simulink model "OMAP"  (R2018b)
settings: Solver=FixedStepDiscrete  StartTime=0.0  StopTime=10.0  FixedStep=0.01  RelTol=1e-3
values from neighbouring files (symbols this model uses):
  Clb_ICADirect_LaneDisp_StateFive = Simulink.Parameter    [omap_ver_442.m]
  Clb_ICADirect_LaneDisp_StateFour = Simulink.Parameter    [omap_ver_442.m]
  Clb_ICADirect_LaneDisp_StateOne = Simulink.Parameter    [omap_ver_442.m]
  Clb_ICADirect_LaneDisp_StateThree = Simulink.Parameter    [omap_ver_442.m]
  Clb_ICADirect_LaneDisp_StateTwo = Simulink.Parameter    [omap_ver_442.m]
  Clb_ICADirect_LaneDisp_StateZero = Simulink.Parameter    [omap_ver_442.m]
  Clb_ICADirect_LaneDispSW = Simulink.Parameter    [omap_ver_442.m]
  Clb_ICADirect_TrnLghtsCom_Switch = Simulink.Parameter    [omap_ver_442.m]
  Clb_ICADirect_TrnLghtsCom_Value = Simulink.Parameter    [omap_ver_442.m]
  Clb_ICADirect_TrnLghtsCrtl_Inhb = Simulink.Parameter    [omap_ver_442.m]
  OMAP_ACCAEB_EMSESC_Decel = Simulink.Parameter    [omap_ver_442.m]
  OMAP_ACCFCW_IC_Decel = Simulink.Parameter    [omap_ver_442.m]
  OMAP_clb_ACC_RVVReqType = Simulink.Parameter    [omap_ver_442.m]
  OMAP_clb_ACC_RVVReqType_Switch = Simulink.Parameter    [omap_ver_442.m]
  OMAP_clb_ACCHeadwayDisplay = Simulink.Parameter    [omap_ver_442.m]
  OMAP_clb_ACCHeadwayDisplay_Switch = Simulink.Parameter    [omap_ver_442.m]
  OMAP_clb_ACCHeadwayIcon = Simulink.Parameter    [omap_ver_442.m]
  OMAP_clb_ACCHeadwayIcon_Switch = Simulink.Parameter    [omap_ver_442.m]
  OMAP_clb_ACCMessagePrompt = Simulink.Parameter    [omap_ver_442.m]
  OMAP_clb_ACCMessagePrompt_Switch = Simulink.Parameter    [omap_ver_442.m]
  OMAP_clb_ACCRequestEPB = Simulink.Parameter    [omap_ver_442.m]
  OMAP_clb_ACCRequestEPB_Switch = Simulink.Parameter    [omap_ver_442.m]
  OMAP_clb_ACCSetSpeed = Simulink.Parameter    [omap_ver_442.m]
  OMAP_clb_ACCSetSpeed_Switch = Simulink.Parameter    [omap_ver_442.m]
  OMAP_clb_ACCSetSpeedDis = Simulink.Parameter    [omap_ver_442.m]
  OMAP_clb_ACCSetSpeedDis_Switch = Simulink.Parameter    [omap_ver_442.m]
  OMAP_clb_ACCState = Simulink.Parameter    [omap_ver_442.m]
  OMAP_clb_ACCState_Switch = Simulink.Parameter    [omap_ver_442.m]
  OMAP_clb_ACCStatusIconDis = Simulink.Parameter    [omap_ver_442.m]
  OMAP_clb_ACCStatusIconDis_Switch = Simulink.Parameter    [omap_ver_442.m]
  OMAP_clb_ACCTorqueReq = Simulink.Parameter    [omap_ver_442.m]
  OMAP_clb_ACCTorqueReq_Switch = Simulink.Parameter    [omap_ver_442.m]
  OMAP_clb_ADAS_State = Simulink.Parameter    [omap_ver_442.m]
  OMAP_clb_ADAS_State_Switch = Simulink.Parameter    [omap_ver_442.m]
  OMAP_clb_AEBAlertReq = Simulink.Parameter    [omap_ver_442.m]
  OMAP_clb_AEBAlertReq_Switch = Simulink.Parameter    [omap_ver_442.m]
  OMAP_clb_AEBBrakingProg = Simulink.Parameter    [omap_ver_442.m]
  OMAP_clb_AEBBrakingProg_Switch = Simulink.Parameter    [omap_ver_442.m]
  OMAP_clb_AEBFaultStatus = Simulink.Parameter    [omap_ver_442.m]
  OMAP_clb_AEBFaultStatus_Switch = Simulink.Parameter    [omap_ver_442.m]
  OMAP_clb_AEBMassageDisp = Simulink.Parameter    [omap_ver_442.m]
  OMAP_clb_AEBMassageDisp_Switch = Simulink.Parameter    [omap_ver_442.m]
  OMAP_clb_AEBState = Simulink.Parameter    [omap_ver_442.m]
  OMAP_clb_AEBState_Switch = Simulink.Parameter    [omap_ver_442.m]
  OMAP_clb_AEBSwitchStatus = Simulink.Parameter    [omap_ver_442.m]
  OMAP_clb_AEBSwitchStatus_Switch = Simulink.Parameter    [omap_ver_442.m]
  OMAP_clb_BrakeRequest = Simulink.Parameter    [omap_ver_442.m]
  OMAP_clb_BrakeRequest_Switch = Simulink.Parameter    [omap_ver_442.m]
  OMAP_clb_DecelerationSet = Simulink.Parameter    [omap_ver_442.m]
  OMAP_clb_DecelerationSet_Switch = Simulink.Parameter    [omap_ver_442.m]
  OMAP_clb_DecelerationType = Simulink.Parameter    [omap_ver_442.m]
  OMAP_clb_DecelerationType_Switch = Simulink.Parameter    [omap_ver_442.m]
  OMAP_clb_DeclControlReq = Simulink.Parameter    [omap_ver_442.m]
  OMAP_clb_DeclControlReq_Switch = Simulink.Parameter    [omap_ver_442.m]
  OMAP_clb_DownorUpGearMinTime = Simulink.Parameter    [omap_ver_442.m]
  OMAP_clb_DownorUpGearMinTime_Switch = Simulink.Parameter    [omap_ver_442.m]
  OMAP_clb_ELKPopupMessage = Simulink.Parameter    [omap_ver_442.m]
  OMAP_clb_ELKPopupMessage_Switch = Simulink.Parameter    [omap_ver_442.m]
  OMAP_clb_ELKSts = Simulink.Parameter    [omap_ver_442.m]
  OMAP_clb_ELKSts_Switch = Simulink.Parameter    [omap_ver_442.m]
  OMAP_clb_ESAFaultSt = Simulink.Parameter    [omap_ver_442.m]
  OMAP_clb_ESAFaultSt_Switch = Simulink.Parameter    [omap_ver_442.m]
  OMAP_clb_ESARequest = Simulink.Parameter    [omap_ver_442.m]
  OMAP_clb_ESARequest_Switch = Simulink.Parameter    [omap_ver_442.m]
  OMAP_clb_ESAState = Simulink.Parameter    [omap_ver_442.m]
  OMAP_clb_ESAState_Switch = Simulink.Parameter    [omap_ver_442.m]
  OMAP_clb_ESATorqueReq = Simulink.Parameter    [omap_ver_442.m]
  OMAP_clb_ESATorqueReq_Switch = Simulink.Parameter    [omap_ver_442.m]
  OMAP_clb_ESCDriveOff = Simulink.Parameter    [omap_ver_442.m]
  OMAP_clb_ESCDriveOff_Switch = Simulink.Parameter    [omap_ver_442.m]
  OMAP_clb_ESCHoldReq = Simulink.Parameter    [omap_ver_442.m]
  OMAP_clb_ESCHoldReq_Switch = Simulink.Parameter    [omap_ver_442.m]
  OMAP_clb_Handsoffwarning = Simulink.Parameter    [omap_ver_442.m]
  OMAP_clb_Handsoffwarning_Switch = Simulink.Parameter    [omap_ver_442.m]
  OMAP_clb_HapticAlarmReq = Simulink.Parameter    [omap_ver_442.m]
  OMAP_clb_HapticAlarmReq_Switch = Simulink.Parameter    [omap_ver_442.m]
  OMAP_clb_HMIPopupMassage = Simulink.Parameter    [omap_ver_442.m]
  OMAP_clb_HMIPopupMassage_Switch = Simulink.Parameter    [omap_ver_442.m]
  OMAP_clb_HWAActionSts = Simulink.Parameter    [omap_ver_442.m]
  OMAP_clb_HWAActionSts_Switch = Simulink.Parameter    [omap_ver_442.m]
  OMAP_clb_HWAMode = Simulink.Parameter    [omap_ver_442.m]
  OMAP_clb_HWAMode_Switch = Simulink.Parameter    [omap_ver_442.m]
  OMAP_clb_HWATurnOnIdctr = Simulink.Parameter    [omap_ver_442.m]
  OMAP_clb_HWATurnOnIdctr_Switch = Simulink.Parameter    [omap_ver_442.m]
  OMAP_clb_ICAMassageDisp = Simulink.Parameter    [omap_ver_442.m]
  OMAP_clb_ICAMassageDisp_Switch = Simulink.Parameter    [omap_ver_442.m]
  OMAP_clb_ICAStatusIcon = Simulink.Parameter    [omap_ver_442.m]
  OMAP_clb_ICAStatusIcon_Switch = Simulink.Parameter    [omap_ver_442.m]
  OMAP_clb_ISLCDriverRemind = Simulink.Parameter    [omap_ver_442.m]
  OMAP_clb_ISLCDriverRemind_Switch = Simulink.Parameter    [omap_ver_442.m]
  OMAP_clb_ISLCState = Simulink.Parameter    [omap_ver_442.m]
  OMAP_clb_ISLCState_Switch = Simulink.Parameter    [omap_ver_442.m]
  OMAP_clb_JAFaultSt = Simulink.Parameter    [omap_ver_442.m]
  OMAP_clb_JAFaultSt_Switch = Simulink.Parameter    [omap_ver_442.m]
  OMAP_clb_LCAPopupMessage = Simulink.Parameter    [omap_ver_442.m]
  OMAP_clb_LCAPopupMessage_Switch = Simulink.Parameter    [omap_ver_442.m]
  OMAP_clb_LCAStatusDisplay = Simulink.Parameter    [omap_ver_442.m]
  OMAP_clb_LCAStatusDisplay_Switch = Simulink.Parameter    [omap_ver_442.m]
  OMAP_clb_LDWStatusDisplay = Simulink.Parameter    [omap_ver_442.m]
  OMAP_clb_LDWStatusDisplay_Switch = Simulink.Parameter    [omap_ver_442.m]
  OMAP_clb_LDWWarningSt = Simulink.Parameter    [omap_ver_442.m]
  OMAP_clb_LDWWarningSt_Switch = Simulink.Parameter    [omap_ver_442.m]
  OMAP_clb_LightControlValid = Simulink.Parameter    [omap_ver_442.m]
  OMAP_clb_LightControlValid_Switch = Simulink.Parameter    [omap_ver_442.m]
  OMAP_clb_LKAActivation = Simulink.Parameter    [omap_ver_442.m]
  OMAP_clb_LKAActivation_Switch = Simulink.Parameter    [omap_ver_442.m]
  OMAP_clb_LKAAngleReq = Simulink.Parameter    [omap_ver_442.m]
  OMAP_clb_LKAAngleReq_Switch = Simulink.Parameter    [omap_ver_442.m]
  OMAP_clb_LKAMode = Simulink.Parameter    [omap_ver_442.m]
  OMAP_clb_LKAMode_Switch = Simulink.Parameter    [omap_ver_442.m]
  OMAP_clb_LKAorELK_CoolTime = Simulink.Parameter    [omap_ver_442.m]
  OMAP_clb_LKAState = Simulink.Parameter    [omap_ver_442.m]
  OMAP_clb_LKAState_Switch = Simulink.Parameter    [omap_ver_442.m]
  OMAP_clb_LKAStatusDisplay = Simulink.Parameter    [omap_ver_442.m]
  OMAP_clb_LKAStatusDisplay_Switch = Simulink.Parameter    [omap_ver_442.m]
  OMAP_clb_LKASwitchState = Simulink.Parameter    [omap_ver_442.m]
  OMAP_clb_LKASwitchState_Switch = Simulink.Parameter    [omap_ver_442.m]
  OMAP_clb_LKATorqFactReq = Simulink.Parameter    [omap_ver_442.m]
  OMAP_clb_LKATorqFactReq_Switch = Simulink.Parameter    [omap_ver_442.m]
  OMAP_clb_PrefillRequest = Simulink.Parameter    [omap_ver_442.m]
  ... (+36 more)
libraries: simulink x184, canmsglib x2
(part 3 of 14)

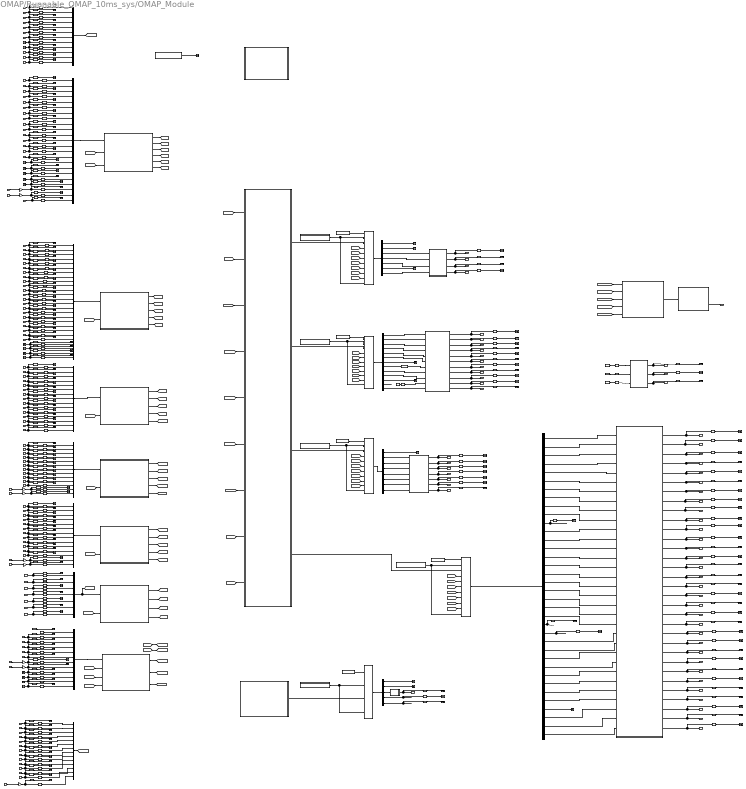
== system OMAP/Runnable_OMAP_10ms_sys/OMAP_Module ==
  note: 暂未参与运算的输出接口
  note: 仲裁#12——ACC单功能调试模式
      | EMS、ESC、EPS、IC：只体现本功能的信号、且其他信号内容强制为“不动作”
  note: 仲裁#17——ESA单功能调试模式
      | EMS、ESC、EPS、IC：只体现本功能的信号、且其他信号内容强制为“不动作”
  note: 仲裁#13——AEB单功能调试模式
      | EMS、ESC、EPS、IC：只体现本功能的信号、且其他信号内容强制为“不动作”
  note: 上面这是版本号
      | 蓝色的子系统是输入，橙色是仲裁输出，
      | 翠绿色的模块是标定量
  note: 仲裁#18——ICA单功能调试模式
      | EMS、ESC：只体现ACC的信号、且其他信号内容强制为“不动作”
      | EPS：只体现本功能的信号、且其他信号内容强制为“不动作”
      | IC：只体现本功能及ACC综合后的的信号、且其他信号内容强制为“不动作”
  note: 仲裁#16——ELK单功能调试模式
      | EMS、ESC、EPS、IC：只体现本功能的信号、且其他信号内容强制为“不动作”
  note: 仲裁#15——LKA单功能调试模式
      | EMS、ESC、EPS、IC：只体现本功能的信号、且其他信号内容强制为“不动作”
  note: 仲裁#14——JA单功能调试模式——
      | EMS、ESC、EPS、IC：只体现本功能的信号、且其他信号内容强制为“不动作”
  FDMMve_d_JaFcnConf : Inport  OutDataTypeStr=uint16
  FDMMve_d_AebFcnConf : Inport  Port=2  OutDataTypeStr=uint16
  FDMMve_d_EsaFcnConf : Inport  Port=3  OutDataTypeStr=uint16
  FDMMve_d_ElkFcnConf : Inport  Port=4  OutDataTypeStr=uint16
  FDMMve_d_LkaFcnConf : Inport  Port=5  OutDataTypeStr=uint16
  FDMMve_d_IcaFcnConf : Inport  Port=6  OutDataTypeStr=uint16
  FDMMve_d_AccFcnConf : Inport  Port=7  OutDataTypeStr=uint16
  FDMMve_d_EwFcnConf : Inport  Port=8  OutDataTypeStr=uint16
  FDMMve_g_Adas2Fapa : Inport  Port=9  OutDataTypeStr=uint32
  FDMMve_d_SignalTStamp : Inport  Port=10  OutDataTypeStr=uint16
  ACCSve_d_ACC_State : Inport  Port=11  OutDataTypeStr=uint16
  ACCSve_g_ACC_TqReq : Inport  Port=12  OutDataTypeStr=single
  ACCSve_d_ACC_TqFlag : Inport  Port=13  OutDataTypeStr=uint16
  ACCSve_g_ACC_DecReq : Inport  Port=14  OutDataTypeStr=single
  ACCSve_d_ACC_DecFlag : Inport  Port=15  OutDataTypeStr=uint16
  ACCSve_d_CIPV_ID : Inport  Port=16  OutDataTypeStr=uint16
  ACCSve_d_ACCActive_Signal : Inport  Port=17  OutDataTypeStr=uint16
  ACCSve_d_ACC_go_request : Inport  Port=18  OutDataTypeStr=uint16
  ACCSve_d_VelocitySet : Inport  Port=19  OutDataTypeStr=uint16
  ACCSve_d_HeadWaySet : Inport  Port=20  OutDataTypeStr=uint16
  ACCSve_d_SignalTStamp : Inport  Port=21  OutDataTypeStr=uint16
  ACCSve_d_ACC_ICA_Flag : Inport  Port=22  OutDataTypeStr=uint16
  ACCSve_d_ACC_ESCDriveOff : Inport  Port=23  OutDataTypeStr=uint16
  ACCSve_d_ACC_ESCHoldReq : Inport  Port=24  OutDataTypeStr=uint16
  ACCSve_d_ACC_EPBReq : Inport  Port=25  OutDataTypeStr=uint16
  ACCSve_d_ACCMessagePrompt : Inport  Port=26  OutDataTypeStr=uint16
  ACCSve_d_ACC_ISLCState : Inport  Port=27  OutDataTypeStr=uint16
  ACCSve_d_ACC_ISLCDriverRemind : Inport  Port=28  OutDataTypeStr=uint16
  AEBSve_d_Prefill_request : Inport  Port=29  OutDataTypeStr=uint16
  AEBSve_d_functionFARCState : Inport  Port=30  OutDataTypeStr=uint16
  AEBSve_g_DecSetpoint : Inport  Port=31  OutDataTypeStr=single
  AEBSve_d_MDDdecRequest : Inport  Port=32  OutDataTypeStr=uint16
  AEBSve_d_MDDdecType : Inport  Port=33  OutDataTypeStr=uint16
  AEBSve_d_ESCDriveOff : Inport  Port=34  OutDataTypeStr=uint16
  AEBSve_d_ESCHoldReq : Inport  Port=35  OutDataTypeStr=uint16
  AEBSve_d_HapticAlarm : Inport  Port=36  OutDataTypeStr=uint16
  AEBSve_d_Braking_progress : Inport  Port=37  OutDataTypeStr=uint16
  AEBSve_d_AEBStatus : Inport  Port=38  OutDataTypeStr=uint16
  AEBSve_d_FCWStatus : Inport  Port=39  OutDataTypeStr=uint16
  AEBSve_d_AEBSwitchStatus : Inport  Port=40  OutDataTypeStr=uint16
  AEBSve_d_AEBFaultStatus : Inport  Port=41  OutDataTypeStr=uint16
  AEBSve_d_AEBAlertReq : Inport  Port=42  OutDataTypeStr=uint16
  AEBSve_d_AEBTips : Inport  Port=43  OutDataTypeStr=uint16
  AEBSve_d_SignalTStamp : Inport  Port=44  OutDataTypeStr=uint16
  AEBSve_d_JABS_AlertSign : Inport  Port=45  OutDataTypeStr=uint16
  AEBSve_d_JABS_SwitchStatus : Inport  Port=46  OutDataTypeStr=uint16
  AEBSve_d_JABS_FltStatus : Inport  Port=47  OutDataTypeStr=uint16
  AEBSve_d_JABS_AlertReq : Inport  Port=48  OutDataTypeStr=uint16
  AEBSve_d_JABS_HapticAlarm : Inport  Port=49  OutDataTypeStr=uint16
  AEBSve_d_JABS_Tips : Inport  Port=50  OutDataTypeStr=uint16
  JABSve_d_DbPrefillReq : Inport  Port=51  OutDataTypeStr=uint16
  JABSve_d_DbFunFARCSta : Inport  Port=52  OutDataTypeStr=uint16
  JABSve_g_DbDecSetpoint : Inport  Port=53  OutDataTypeStr=single
  JABSve_d_DbMDDdecRequest : Inport  Port=54  OutDataTypeStr=uint16
  JABSve_d_DbMDDdecType : Inport  Port=55  OutDataTypeStr=uint16
  JABSve_d_DbHapticAlarm : Inport  Port=56  OutDataTypeStr=uint16
  JABSve_d_DbBraking_progress : Inport  Port=57  OutDataTypeStr=uint16
  JABSve_d_DbSignalTStamp : Inport  Port=58  OutDataTypeStr=uint16
  JABSve_d_DbJACWStatus : Inport  Port=59  OutDataTypeStr=uint16
  JABSve_d_DbSwitchStatus : Inport  Port=60  OutDataTypeStr=uint16
  JABSve_d_DbFltStatus : Inport  Port=61  OutDataTypeStr=uint16
  JABSve_d_DbAlertReq : Inport  Port=62  OutDataTypeStr=uint16
  JABSve_d_DbTips : Inport  Port=63  OutDataTypeStr=uint16
  JABSve_d_DbESCDriveOff : Inport  Port=64  OutDataTypeStr=uint16
  JABSve_d_DbESCHoldReq : Inport  Port=65  OutDataTypeStr=uint16
  LKASve_y_Vehicle_Lane_Display : Inport  Port=66  OutDataTypeStr=uint8
  LKASve_y_LDW_Status_Display : Inport  Port=67  OutDataTypeStr=uint8
  LKASve_y_LKA_Status_Display : Inport  Port=68  OutDataTypeStr=uint8
  LKASve_y_LDW_Flag : Inport  Port=69  OutDataTypeStr=uint8
  LKASve_y_Hands_Off_Warning : Inport  Port=70  OutDataTypeStr=uint8
  LKASve_y_LKA_Action_Indication : Inport  Port=71  OutDataTypeStr=uint8
  LKASve_y_HMI_Popup_Status : Inport  Port=72  OutDataTypeStr=uint8
  LKASve_y_EPS_State_Control : Inport  Port=73  OutDataTypeStr=uint8
  LKASve_g_LKA_SWA_Control : Inport  Port=74  OutDataTypeStr=single
  LKASve_g_EPS_Factor_Control : Inport  Port=75  OutDataTypeStr=single
  LKASve_y_EPS_LKA_Control : Inport  Port=76  OutDataTypeStr=uint8
  LKASve_y_LKATorqueReq : Inport  Port=77  OutDataTypeStr=uint8
  LKASve_g_LKATorqueReq_Value : Inport  Port=78  OutDataTypeStr=single
  ELKSve_y_state_ELK_function : Inport  Port=79  OutDataTypeStr=uint8
  ELKSve_y_ELK_HapticAlarmReq : Inport  Port=80  OutDataTypeStr=uint8
  ELKSve_y_Hands_Off_Warning : Inport  Port=81  OutDataTypeStr=uint8
  ELKSve_y_ELK_Action_Indication : Inport  Port=82  OutDataTypeStr=uint8
  ELKSve_y_HMI_Popup_Status : Inport  Port=83  OutDataTypeStr=uint8
  ELKSve_y_EPS_State_Control : Inport  Port=84  OutDataTypeStr=uint8
  ELKSve_g_ELK_SWA_Control : Inport  Port=85  OutDataTypeStr=single
  ELKSve_g_EPS_Factor_Control : Inport  Port=86  OutDataTypeStr=single
  ELKSve_y_EPS_ELK_Control : Inport  Port=87  OutDataTypeStr=uint8
  ELKSve_y_ELK_VehicleLaneDisp : Inport  Port=88  OutDataTypeStr=uint8
  ELKSve_y_ELK_ELKSts : Inport  Port=89  OutDataTypeStr=uint8
  ELKSve_y_SignalTStamp : Inport  Port=90  OutDataTypeStr=uint8
  ELKSve_y_LKATorqueReq : Inport  Port=91  OutDataTypeStr=uint8
  ELKSve_g_LKATorqueReq_Value : Inport  Port=92  OutDataTypeStr=single
  ICABve_d_SignalTStamp : Inport  Port=93  OutDataTypeStr=uint16
  ICABva_d_ICAB2HMI : Inport  Port=94  OutDataTypeStr=uint16
  ICABve_g_SteerAngleCmd : Inport  Port=95  OutDataTypeStr=single
  ICABve_d_ICAMode : Inport  Port=96  OutDataTypeStr=uint16
  ICABve_d_ICAState : Inport  Port=97  OutDataTypeStr=uint16
  ICABve_d_LKATorqueReq : Inport  Port=98  OutDataTypeStr=uint16
  ICABve_g_LKATorqueReq_Value : Inport  Port=99  OutDataTypeStr=single
  IMAPve_d_EPS_LKA_State : Inport  Port=100  OutDataTypeStr=uint16
  IMAPve_g_ESC_LonAcc : Inport  Port=101  OutDataTypeStr=single
  IMAPva_d_obj_id : Inport  Port=102  OutDataTypeStr=uint16
  IMAPva_g_obj_pos_x : Inport  Port=103  OutDataTypeStr=single
  IMAPve_d_ESC_Veh_Standstill : Inport  Port=104  OutDataTypeStr=uint16
  IMAPve_g_L0_C0 : Inport  Port=105  OutDataTypeStr=single
  IMAPve_g_L0_C1 : Inport  Port=106  OutDataTypeStr=single
  IMAPve_g_L0_C2 : Inport  Port=107  OutDataTypeStr=single
  IMAPve_g_L0_C3 : Inport  Port=108  OutDataTypeStr=single
  IMAPve_g_R0_C0 : Inport  Port=109  OutDataTypeStr=single
  IMAPve_g_R0_C1 : Inport  Port=110  OutDataTypeStr=single
  IMAPve_g_R0_C2 : Inport  Port=111  OutDataTypeStr=single
  IMAPve_g_R0_C3 : Inport  Port=112  OutDataTypeStr=single
  IMAPve_d_APA_AutoPark_WorkSt : Inport  Port=113  OutDataTypeStr=uint16
  ESASve_y_ESA_State : Inport  Port=114  OutDataTypeStr=uint8
  ESASve_g_ESA_SWA_CMD : Inport  Port=115  OutDataTypeStr=single
  ESASve_g_EPS_Factor_Control : Inport  Port=116  OutDataTypeStr=single
  ESASve_y_ESA_FaultSt : Inport  Port=117  OutDataTypeStr=uint8
  ESASve_y_ESARequest : Inport  Port=118  OutDataTypeStr=uint8
  ESASve_y_ESATorqueReq : Inport  Port=119  OutDataTypeStr=single
  ESASve_y_LKAActivation : Inport  Port=120  OutDataTypeStr=uint8
  ACCS_Direct : Subsystem
  AEBS_Direct : Subsystem
  Bus Creator : BusCreator  Inputs=7
  Bus Selector : BusSelector  OutputSignals=OMAPve_y_ACC_Engine_Start_Request_1,OMAPve_g_PotACCTqReq_1,OMAPve_g_ACCTqReq_1,OMAPve_y_Powertrain_torquewheel_request_1,OMAPve_g_TminUp_or_downGear_1,OMAPve_y_stAcvTqWhlPTPotReq_1,OMAPve_y_Function_Acc_status_1
  Bus Selector1 : BusSelector  OutputSignals=OMAPve_g_Deceleration_setpoint_device_1,OMAPve_y_MDD_Decelerationcontrol_request_1,OMAPve_y_Prefill_request_1,OMAPve_y_ADAS_ESCDriveOff,OMAPve_y_ADAS_ESCHoldReq,OMAPve_y_MDD_deceleration_type_1,OMAPve_y_State_of_the_functionFARC_det_1,OMAPve_y_AEB_Status_1,OMAPve_y_Decel_Request_1,OMAPve_y_AEB_Braking_progress_1,OMAPve_y_FCW_Status_1,OMAPve_y_Haptic_Alarm_1,OMAPve_y_ADAS_ACCRequestEPB
  Bus Selector2 : BusSelector  OutputSignals=OMAPve_y_Power_steering_power_cut3F2_2,OMAPve_y_General_state_of_LKA_function3F2_2,OMAPve_g_Coefficient_toregulate_EPS_2,OMAPve_g_Column_angle_setpoint3F2_2,OMAPve_y_Permit_to_know_if_LKA_or_LPA3F2_2,OMAPve_y_ADAS_ESAState_2,OMAPve_g_ADAS_ESATorqueReq_2,OMAPve_y_ADAS_ESARequest_2
  Bus Selector3 : BusSelector  OutputSignals=OMAPve_y_ADAS_ELKPopupMessage_2,OMAPve_y_ADAS_ESAFaultSt_2,OMAPve_y_ADAS_HWAMode_2,OMAPve_y_ADAS_HWATurnOnIndicator_2,OMAPve_y_ADAS_HWAActionSts_2,OMAPve_y_ADAS_LightControlValid_2,OMAPve_y_ADAS_ISLCState_2,OMAPve_y_ADAS_ISLCDriverRemind_2,OMAPve_y_ADAS_TurnLightsCommand_2,OMAPve_y_ADAS_JAFaultSt_2,OMAPve_y_TSR_Vision_Only_Sign_Type_2,OMAPve_y_ACC_DesiredHeadway_Display_2,OMAPve_y_ACC_DesiredHeadway_Icon_Basic_2,OMAPve_y_ACC_Desired_Set_Speed_2,OMAPve_y_ACC_Set_Speed_Display_2,OMAPve_y_ACC_Vehicle_Icon_Display_2,OMAPve_y_RVVACC_Vehiclespeed_request_type_2,OMAPve_y_ACC_Pop_Up_Message_2,OMAPve_y_AEB_Alert_Req_2,OMAPve_y_AEB_Fault_Status_2,OMAPve_y_AEB_Switch_Status_2,OMAPve_y_AEB_tips_2,OMAPve_y_ACC_HMI_TgtDisp_Flag_2,OMAPve_y_TARGET_POSITION_2,OMAPve_y_Hands_off_warning_2,OMAPve_y_HMI_Popup_Status_2,OMAPve_y_Vehicle_Lane_Display_2,OMAPve_y_LDW_Flag_2,OMAPve_y_LDW_Status_Display_2,OMAPve_y_LKA_Mode_from_Camera_2,OMAPve_y_LKA_Status_Display_2,OMAPve_y_LKA_Switch_State_2,OMAPve_y_LKA_action_indication_2,OMAPve_y_ADAS_ELKSts_2,OMAPve_y_ICA_HMI_Txt_Disp_2,OMAPve_y_TJA_status_icon_2
  Bus Selector4 : BusSelector  OutputSignals=OMAPve_y_ABS_ESP_power_cut_request2_2,OMAPve_y_ASR_connection_dis_demand2_2,OMAPve_y_TYPE_RAPPORT_2,OMAPve_y_ECU_operating_phase_2,OMAPve_y_Radar_State_2
  Bus_ACCS : BusCreator  Inputs=23
  Bus_AEBS : BusCreator  Inputs=26
  Bus_ELKS : BusCreator  Inputs=14
  Bus_FDMM : BusCreator  Inputs=12
  Bus_ICA : BusCreator  Inputs=12
  Bus_IMAP : BusCreator  Inputs=14
  Bus_JABS : BusCreator  Inputs=15
  Bus_LKAS : BusCreator  Inputs=13
  CAN Pack : canmsglib/CAN Pack  CANdbFile=E:\DATA\L3_Work\信号矩阵+DBC\DBC\Observe_OMAP.dbc  MsgList=OMAPve_g_ob019L_100  MsgName=OMAPve_g_ob019L_100  MsgIDType=Standard (11-bit identifier)  MsgIdentifier=1136  MsgLength=8  SignalInfo=ob_AEBarbJADecReq$39$1$2$2$1$0$1$0$-Inf$Inf$#ob_AEBarbJADecSet$40$8$2$2$1$0$5.000000e-02$-1.065000e+01$-Inf$Inf$#ob_AEBarbJADecType$37$2$2$2$1$0$1$0$-Inf$Inf$#ob_isJAorDeepAEB$36$1$2$2$1$0$1$0$-Inf$Inf$#ob_isLowACCandLowAEB$35$1$2$2$1$0$1$0$-Inf$Inf$#  NSignals=5  StartBits=str2num('[int32(39);int32(40);int32(37);int32(36);int32(35)]')  SignalSizes=str2num('[int32(1);int32(8);int32(2);int32(1);int32(1)]')  ByteOrders=str2num('[int32(2);int32(2);int32(2);int32(2);int32(2)]')  DataTypes=str2num('[int32(2);int32(2);int32(2);int32(2);int32(2)]')  MultiplexTypes=str2num('[int32(1);int32(1);int32(1);int32(1);int32(1)]')  MultiplexValues=str2num('[double(0);double(0);double(0);double(0);double(0)]')  Factors=str2num('[double(1);double(5.000000e-02);double(1);double(1);double(1)]')  Offsets=str2num('[double(0);double(-1.065000e+01);double(0);double(0);double(0)]')  Minimums=str2num('[double(-Inf);double(-Inf);double(-Inf);double(-Inf);double(-Inf)]')  Maximums=str2num('[double(Inf);double(Inf);double(Inf);double(Inf);double(Inf)]')  Remote=off  ApplyMinMax=off  BusOutput=off
      settings: SourceProductName=Simulink Real-Time  SourceProductBaseCode=XP  DataFormat=CANdb specified signals
  CAN Unpack : canmsglib/CAN Unpack  MsgList=(none)  MsgName=CAN Msg  MsgIDType=Standard (11-bit identifier)  MsgIdentifier=1136  MsgLength=8  SignalInfo=ob019H$24$32$2$2$1$0$1$0$-Inf$Inf$#ob019L$56$32$2$2$1$0$1$0$-Inf$Inf$#  NSignals=2  IDPort=off  TimestampPort=off  ErrorPort=off  RemotePort=off  LengthPort=off  StatusPort=off  StartBits=str2num('[int32(24);int32(56)]')  SignalSizes=str2num('[int32(32);int32(32)]')  ByteOrders=str2num('[int32(2);int32(2)]')  DataTypes=str2num('[int32(2);int32(2)]')  MultiplexTypes=str2num('[int32(1);int32(1)]')  MultiplexValues=str2num('[double(0);double(0)]')  Factors=str2num('[double(1);double(1)]')  Offsets=str2num('[double(0);double(0)]')  Minimums=str2num('[double(-Inf);double(-Inf)]')  Maximums=str2num('[double(Inf);double(Inf)]')  ApplyMinMax=off
      settings: SourceProductName=Simulink Real-Time  SourceProductBaseCode=XP
  Calib : Subsystem
  Constant : Constant  Value=OMAP_Switch_EMS  OutDataTypeStr=uint8
  Constant1 : Constant  Value=OMAP_Switch_ESC  OutDataTypeStr=uint8
  Constant2 : Constant  Value=OMAP_Switch_EPS  OutDataTypeStr=uint8
  Constant3 : Constant  Value=OMAP_Switch_IC  OutDataTypeStr=uint8
  Constant4 : Constant  Value=OMAP_Switch_OTHER  OutDataTypeStr=uint8
  Constant6 : Constant  Value=442  OutDataTypeStr=uint16
  Constant7 : Constant  Value=0  OutDataTypeStr=uint8
  Data Type Conversion{,1..10,13..21,23..32,37..38,43..45,52..53,55,57..58,60,62..63,78..86,89..91,93,95..98,100,149..160,162..165,167..177,180} (89 alike) : DataTypeConversion  OutDataTypeStr=uint16
  Data Type Conversion{34..35,40,46..47,50,54,56,88,92,94,99,101..110,144..145,161,166,179,182} (28 alike) : DataTypeConversion  OutDataTypeStr=single
  Data Type Conversion{11..12,33,36,39,41..42,48..49,51,87,111..119,139..143,146..148,178} (29 alike) : DataTypeConversion  OutDataTypeStr=uint8
  Data Type Conversion22 : DataTypeConversion  OutDataTypeStr=uint32
  Default_EMS : Subsystem
  Default_EPS : Subsystem
  Default_ESC : Subsystem
  Default_IC : Subsystem
  Default_OTHER : Subsystem
  ELKS_Direct : Subsystem
  ESAS_Direct : Subsystem
  Gain{,1,6..12} (9 alike) : Gain
  Ground{,1..14} (15 alike) : Ground
  ICA_Direct_G59 : Subsystem
  Index Vector{,1..3} (4 alike) : MultiPortSwitch  DataPortOrder=Zero-based contiguous  Inputs=10  zeroidx=on
  Index Vector4 : MultiPortSwitch  DataPortOrder=Zero-based contiguous  zeroidx=on
  JABS_Direct : Subsystem
  LKAS_Direct : Subsystem
  OMAPve_y_ADAS_LCAPopupMessage1 : Constant  Value=0  OutDataTypeStr=uint8
  OMAPve_y_ADAS_LCAStatusDisplay1 : Constant  Value=0  OutDataTypeStr=uint8
  OMAPve_y_ADAS_State1 : Constant  Value=0  OutDataTypeStr=uint8
  OTHER_Default_Arbitration : Subsystem
  Subsystem : Subsystem
  Subsystem1 : Subsystem
  Subsystem2 : Subsystem
  Subsystem3 : Subsystem
  Subsystem4 : Subsystem
  Subsystem6 : Subsystem
  Subsystem7 : Subsystem
  Subsystem8 : Subsystem
  Terminator{,1..9} (10 alike) : Terminator
  ob_In_convert{1..10,12..13,15,17..29,31..51,53..64,88..90,92..97,117,119,121,130..138,143} (81 alike) : DataTypeConversion  OutDataTypeStr=uint16
  ob_In_convert11 : DataTypeConversion  OutDataTypeStr=uint32
  ob_In_convert{14,16,30,52,73..74,82..83,91,118,120,122..129,140,142,144} (22 alike) : DataTypeConversion  OutDataTypeStr=single
  ob_In_convert{65..72,75..81,84..87,139,141} (21 alike) : DataTypeConversion  OutDataTypeStr=uint8
  ob_In_terminator{1..105,117..144,149..151} (136 alike) : Terminator
  ob_convert{1,6..20,24,26..27,29..49,52..53,55..63,65..67,70,72..73,164..165,172,178} (61 alike) : DataTypeConversion  OutDataTypeStr=uint8
  ob_convert{23,25,28,50..51,54} (6 alike) : DataTypeConversion  OutDataTypeStr=single
  ob_terminator{1,6..20,23..64,66..67,70,72..73} (63 alike) : Terminator
  OMAPve_y_ADAS_ISLCState : Outport
  OMAPve_y_ADAS_ISLCDriverRemind : Outport  Port=2
  OMAPve_y_ADAS_ACCHeadwayDisplay : Outport  Port=3
  OMAPve_y_ADAS_ACCHeadwayIcon : Outport  Port=4
  OMAPve_y_ADAS_ACCSetSpeed : Outport  Port=5
  OMAPve_y_ADAS_ACCSetSpeedDis : Outport  Port=6
  OMAPve_y_ADAS_ACCStatusIconDis : Outport  Port=7
  OMAPve_y_ADAS_ACC_RVVReqType : Outport  Port=8
  OMAPve_y_ADAS_ACCMessagePrompt : Outport  Port=9
      settings: AttributesFormatString=%<Description>在G59值的定义变了
  OMAPve_y_ADAS_AEBAlertReq : Outport  Port=10
      settings: AttributesFormatString=%<Description>在G59新增了值3：JA报警
  OMAPve_y_ADAS_AEBFaultStatus : Outport  Port=11
  OMAPve_y_ADAS_AEBSwitchStatus : Outport  Port=12
  OMAPve_y_ADAS_AEBMassageDisp : Outport  Port=13
  OMAPve_g_ADAS_ACCTorqueReq : Outport  Port=14
  OMAPve_y_ADAS_TorqueActivReq : Outport  Port=15
  OMAPve_g_ADAS_DownorUpGearMinTime : Outport  Port=16
  OMAPve_y_ADAS_UpDownGearChange : Outport  Port=17
  OMAPve_y_ADAS_ACCState : Outport  Port=18
  OMAPve_g_ADAS_DecelerationSet : Outport  Port=19
  OMAPve_y_ADAS_DeclControlReq : Outport  Port=20
  OMAPve_y_ADAS_PrefillRequest : Outport  Port=21
  OMAPve_y_ADAS_ESCDriveOff : Outport  Port=22
  OMAPve_y_ADAS_ESCHoldReq : Outport  Port=23
  OMAPve_y_ADAS_DecelerationType : Outport  Port=24
  OMAPve_y_ADAS_AEBState : Outport  Port=25
      settings: AttributesFormatString=%<Description>在G59值的定义改变
  OMAPve_y_ADAS_BrakeRequest : Outport  Port=26
  OMAPve_y_ADAS_AEBBrakingProg : Outport  Port=27
  OMAPve_y_ADAS_HapticAlarmReq : Outport  Port=28
  OMAPve_y_ADAS_Handsoffwarning : Outport  Port=29
  OMAPve_y_ADAS_HMIPopupMassage : Outport  Port=30
  OMAPve_y_ADAS_VehicleLaneDisp : Outport  Port=31
      settings: AttributesFormatString=%<Description>在G59值的定义变了
  OMAPve_y_ADAS_LDWWarningSt : Outport  Port=32
  OMAPve_y_ADAS_LDWStatusDisplay : Outport  Port=33
  OMAPve_y_ADAS_LKAMode : Outport  Port=34
  OMAPve_y_ADAS_LKAStatusDisplay : Outport  Port=35
  OMAPve_y_ADAS_LKASwitchState : Outport  Port=36
  OMAPve_y_ADAS_ELKSts : Outport  Port=37
  OMAPve_y_ADAS_LCAStatusDisplay : Outport  Port=38
  OMAPve_y_ADAS_LCAPopupMessage : Outport  Port=39
  OMAPve_y_ADAS_LKAState : Outport  Port=40
      settings: AttributesFormatString=%<Description>在G59改了信号周期。内容没变
  OMAPve_g_ADAS_LKATorqFactReq : Outport  Port=41
      settings: AttributesFormatString=%<Description>在G59改了信号周期。内容没变
  OMAPve_g_ADAS_LKAAngleReq : Outport  Port=42
      settings: AttributesFormatString=%<Description>在G59改了信号周期。内容没变
  OMAPve_y_ADAS_LKAActivation : Outport  Port=43
  OMAPve_y_ADAS_ESAState : Outport  Port=44
  OMAPve_g_ADAS_ESATorqueReq : Outport  Port=45
  OMAPve_y_ADAS_ESARequest : Outport  Port=46
  OMAPve_y_ADAS_ICAMassageDisp : Outport  Port=47
      settings: AttributesFormatString=%<Description>在G59值的定义变了
  OMAPve_y_ADAS_ICAStatusIcon : Outport  Port=48
  OMAPve_y_ADAS_HWAMode : Outport  Port=49
  OMAPve_y_ADAS_HWATurnOnIdctr : Outport  Port=50
  OMAPve_y_ADAS_ESAFaultSt : Outport  Port=51
  OMAPve_y_ADAS_JAFaultSt : Outport  Port=52
  OMAPve_y_ADAS_HWAActionSts : Outport  Port=53
  OMAPve_y_ADAS_ACCRequestEPB : Outport  Port=54
  OMAPve_y_ADAS_State : Outport  Port=55
  OMAPve_y_ADAS_LightControlValid : Outport  Port=56
  OMAPve_g_ob019L_100 : Outport  Port=57
  OMAPve_y_ADAS_ELKPopupMessage : Outport  Port=58
  OMAPve_y_ADAS_TurnLightsCommand : Outport  Port=59
  wires:
  OMAPve_y_ADAS_LCAStatusDisplay1/1 -> ob_convert164/1
  OMAPve_y_ADAS_LCAPopupMessage1/1 -> ob_convert165/1
  OMAPve_y_ADAS_State1/1 -> ob_convert178/1
  AEBS_Direct/5(AEB_Input) -> [AEB_Input]
  AEBS_Direct/3(AEB_EPS) -> [AEB_EPS]
  Subsystem6/31(Out31) -> OMAPve_y_ADAS_ICAMassageDisp/1, ob_convert56/1
  Bus Selector1/11 -> Terminator5/1  "<OMAPve_y_FCW_Status_1>"
  [AEB_IC] -> Index Vector3/5
  Bus Selector/6 -> Terminator3/1  "<OMAPve_y_stAcvTqWhlPTPotReq_1>"
  ICA_Direct_G59/3(ICA_Input) -> [ICA_Input]
  Subsystem2/2(Out2) -> ob_convert24/1, OMAPve_y_ADAS_TorqueActivReq/1
  Bus Selector/2 -> Terminator2/1  "<OMAPve_g_PotACCTqReq_1>"
  ELKS_Direct/3(ELK_EPS) -> [ELK_EPS]
  [LKA_EMS] -> Index Vector/7
  Subsystem/1(Out1) -> Index Vector/3
  [LKA_EPS] -> Index Vector2/7
  Index Vector4/1 -> Bus Selector4/1
  ICA_Direct_G59/2(ICA_IC) -> [ICA_IC]
  Subsystem6/11(Out11) -> OMAPve_y_ADAS_ACCHeadwayDisplay/1, ob_convert8/1
  Subsystem3/3(Out3) -> ob_convert30/1, OMAPve_y_ADAS_PrefillRequest/1
  [ELK_EMS] -> Index Vector/8
  Default_OTHER/1(Default) -> Index Vector4/4, Index Vector4/2
  Constant/1 -> Index Vector/1  "Switch_EMS"
  ELKS_Direct/4(ELK_IC) -> [ELK_IC]
  AEBS_Direct/4(AEB_IC) -> [AEB_IC]
  Bus Selector3/23 -> ob_convert19/1  "<OMAPve_y_ACC_HMI_TgtDisp_Flag_2>"
  Subsystem6/21(Out21) -> ob_convert18/1, OMAPve_y_ADAS_AEBMassageDisp/1
  [JA_EPS] -> Index Vector2/6
  Constant4/1 -> Index Vector4/1  "Switch"
  AEBS_Direct/2(AEB_ESC) -> [AEB_ESC]
  Subsystem8/1(Out1) -> ob_convert26/1, OMAPve_y_ADAS_UpDownGearChange/1
  [FD_Input] -> LKAS_Direct/2(Input_FDMM)
  [ELK_EPS] -> Index Vector2/8
  LKAS_Direct/1(LKA_EMS) -> [LKA_EMS]
  LKAS_Direct/3(LKA_EPS) -> [LKA_EPS]
  [AEB_EPS] -> Index Vector2/5
  [ACC_EPS] -> Index Vector2/4
  ESAS_Direct/4(ESA_IC) -> [ESA_IC]
  Subsystem6/26(Out26) -> OMAPve_y_ADAS_LDWStatusDisplay/1, ob_convert42/1
  Subsystem6/28(Out28) -> ob_convert44/1, OMAPve_y_ADAS_LKAStatusDisplay/1
  Subsystem4/4(Out4) -> ob_convert52/1, OMAPve_y_ADAS_LKAActivation/1
  Subsystem6/29(Out29) -> OMAPve_y_ADAS_LKASwitchState/1, ob_convert45/1
  Subsystem4/3(Out3) -> ob_convert51/1, OMAPve_g_ADAS_LKAAngleReq/1
  Subsystem4/2(Out2) -> ob_convert50/1, OMAPve_g_ADAS_LKATorqFactReq/1
  [ESA_EPS] -> Index Vector2/9
  Subsystem6/12(Out12) -> OMAPve_y_ADAS_ACCHeadwayIcon/1, ob_convert9/1
  Subsystem3/6(Out6) -> ob_convert33/1, OMAPve_y_ADAS_DecelerationType/1
  Subsystem/2(Out2) -> Index Vector1/3
  Bus Selector1/7 -> Terminator4/1  "<OMAPve_y_State_of_the_functionFARC_det_1>"
  Default_EPS/1(Default_EPS) -> Index Vector2/11, Index Vector2/2
  Subsystem6/15(Out15) -> OMAPve_y_ADAS_ACCStatusIconDis/1, ob_convert12/1
  Subsystem6/32(Out32) -> OMAPve_y_ADAS_ICAStatusIcon/1, ob_convert57/1
  [ESA_EMS] -> Index Vector/9
  ACCS_Direct/6(ACC_to_ICA) -> [ACC_to_ICA]
  [AEB_ESC] -> Index Vector1/5
  ACCS_Direct/1(ACC_EMS) -> [ACC_EMS]
  Subsystem6/27(Out27) -> OMAPve_y_ADAS_LKAMode/1, ob_convert43/1
  Subsystem/3(Out3) -> Index Vector2/3
  [JA_IC] -> Index Vector3/6
  [FD_Input] -> ESAS_Direct/2(Input_FDMM)
  Bus Selector4/2 -> Terminator9/1  "<OMAPve_y_ASR_connection_dis_demand2_2>"
  Bus Selector3/24 -> ob_convert20/1  "<OMAPve_y_TARGET_POSITION_2>"
  JABS_Direct/1(JA_EMS) -> [JA_EMS]
  [FD_Input] -> ELKS_Direct/2(Input_FDMM)
  [ACC_ESC] -> [ICA_ESC]
  Bus Selector/1 -> Terminator1/1  "<OMAPve_y_ACC_Engine_Start_Request_1>"
  Bus Selector3/33 -> Terminator7/1  "<OMAPve_y_LKA_action_indication_2>"
  Constant1/1 -> Index Vector1/1  "Switch_ESC"
  Subsystem6/24(Out24) -> OMAPve_y_ADAS_VehicleLaneDisp/1, ob_convert40/1
  ESAS_Direct/1(ESA_EMS) -> [ESA_EMS]
  [ACC_EMS] -> Index Vector/4
  Subsystem6/14(Out14) -> OMAPve_y_ADAS_ACCSetSpeedDis/1, ob_convert11/1
  Bus Selector2/1 -> Terminator6/1  "<OMAPve_y_Power_steering_power_cut3F2_2>"
  ACCS_Direct/4(ACC_IC) -> [ACC_IC]
  Subsystem2/3(Out3) -> ob_convert25/1, OMAPve_g_ADAS_DownorUpGearMinTime/1
  Default_ESC/1(Default_ESC) -> Index Vector1/11, Index Vector1/2
  ELKS_Direct/1(ELK_EMS) -> [ELK_EMS]
  Subsystem2/4(Out4) -> OMAPve_y_ADAS_ACCState/1, ob_convert27/1
  [ACC_EMS] -> [ICA_EMS]
  JABS_Direct/4(JA_IC) -> [JA_IC]
  Subsystem3/8(Out8) -> OMAPve_y_ADAS_BrakeRequest/1, ob_convert35/1
  [LKA_IC] -> Index Vector3/7
  JABS_Direct/2(JA_ESC) -> [JA_ESC]
  [JA_ESC] -> Index Vector1/6
  Subsystem6/17(Out17) -> ob_convert14/1, OMAPve_y_ADAS_ACCMessagePrompt/1
  [AEB_EMS] -> Index Vector/5
  Bus Selector4/4 -> ob_convert63/1  "<OMAPve_y_ECU_operating_phase_2>"
  Subsystem3/2(Out2) -> OMAPve_y_ADAS_DeclControlReq/1, ob_convert29/1
  Bus Selector4/1 -> Terminator8/1  "<OMAPve_y_ABS_ESP_power_cut_request2_2>"
  Subsystem6/19(Out19) -> ob_convert16/1, OMAPve_y_ADAS_AEBFaultStatus/1
  Subsystem3/9(Out9) -> OMAPve_y_ADAS_AEBBrakingProg/1, ob_convert36/1
  [ICA_EMS] -> Index Vector/10
  [ACC_ESC] -> Index Vector1/4
  ELKS_Direct/5(ELK_Input) -> [ELK_Input]
  Subsystem6/20(Out20) -> ob_convert17/1, OMAPve_y_ADAS_AEBSwitchStatus/1
  LKAS_Direct/5(LKA_Input) -> [LKA_Input]
  [JA_EMS] -> Index Vector/6
  ESAS_Direct/3(ESA_EPS) -> [ESA_EPS]
  Subsystem3/1(Out1) -> OMAPve_g_ADAS_DecelerationSet/1, ob_convert28/1
  [ICA_ESC] -> Index Vector1/10
  Subsystem6/16(Out16) -> OMAPve_y_ADAS_ACC_RVVReqType/1, ob_convert13/1
  LKAS_Direct/2(LKA_ESC) -> [LKA_ESC]
  ICA_Direct_G59/1(ICA_EPS) -> [ICA_EPS]
  Subsystem/4(Out4) -> Index Vector3/3
  Bus Selector4/5 -> ob_convert66/1  "<OMAPve_y_Radar_State_2>"
  JABS_Direct/3(JA_EPS) -> [JA_EPS]
  Subsystem6/22(Out22) -> OMAPve_y_ADAS_Handsoffwarning/1, ob_convert38/1
  AEBS_Direct/1(AEB_EMS) -> [AEB_EMS]
  ELKS_Direct/2(ELK_ESC) -> [ELK_ESC]
  JABS_Direct/5(JA_Input) -> [JA_Input]
  ACCS_Direct/3(ACC_EPS) -> [ACC_EPS]
  Subsystem6/25(Out25) -> OMAPve_y_ADAS_LDWWarningSt/1, ob_convert41/1
  Constant3/1 -> Index Vector3/1  "Switch_IC"
  [ELK_ESC] -> Index Vector1/8
  [ESA_ESC] -> Index Vector1/9
  Subsystem6/13(Out13) -> OMAPve_y_ADAS_ACCSetSpeed/1, ob_convert10/1
  Index Vector1/1 -> Bus Selector1/1
  Index Vector/1 -> Bus Selector/1
  Constant6/1 -> Terminator/1  "ob_OMAP_version"
  [ACC_IC] -> Index Vector3/4
  ACCS_Direct/5(ACC_Input) -> [ACC_Input]
  LKAS_Direct/4(LKA_IC) -> [LKA_IC]
  Index Vector3/1 -> Bus Selector3/1
  Subsystem6/23(Out23) -> OMAPve_y_ADAS_HMIPopupMassage/1, ob_convert39/1
  [LKA_ESC] -> Index Vector1/7
  Subsystem6/18(Out18) -> ob_convert15/1, OMAPve_y_ADAS_AEBAlertReq/1
  ACCS_Direct/2(ACC_ESC) -> [ACC_ESC]
  Index Vector2/1 -> Bus Selector2/1
  Bus Selector3/11 -> ob_convert1/1  "<OMAPve_y_TSR_Vision_Only_Sign_Type_2>"
  ESAS_Direct/2(ESA_ESC) -> [ESA_ESC]
  Subsystem2/1(Out1) -> OMAPve_g_ADAS_ACCTorqueReq/1, ob_convert23/1
  Subsystem4/1(Out1) -> ob_convert49/1, OMAPve_y_ADAS_LKAState/1
  Constant2/1 -> Index Vector2/1  "Switch_EPS"
  OTHER_Default_Arbitration/1(Arbitration) -> Index Vector4/3
  Subsystem6/30(Out30) -> OMAPve_y_ADAS_ELKSts/1, ob_convert46/1
  Subsystem3/5(Out5) -> OMAPve_y_ADAS_ESCHoldReq/1, ob_convert32/1
  Subsystem3/4(Out4) -> ob_convert31/1, OMAPve_y_ADAS_ESCDriveOff/1
  Subsystem3/11(Out11) -> ob_convert67/1, OMAPve_y_ADAS_ACCRequestEPB/1
  ob_convert1/1 -> ob_terminator1/1  "ob_OMAPve_y_ADAS_TSRSignType"
  ob_convert6/1 -> ob_terminator6/1  "ob_OMAPve_y_ADAS_ISLCState"
  ob_convert7/1 -> ob_terminator7/1  "ob_OMAPve_y_ADAS_ISLCDriverRmd"
  ob_convert8/1 -> ob_terminator8/1  "ob_OMAPve_y_ADAS_ACCHeadwayDisp"
  ob_convert9/1 -> ob_terminator9/1  "ob_OMAPve_y_ADAS_ACCHeadwayIcon"
  ob_convert10/1 -> ob_terminator10/1  "ob_OMAPve_y_ADAS_ACCSetSpeed"
  ob_convert11/1 -> ob_terminator11/1  "ob_OMAPve_y_ADAS_ACCSetSpeedDis"
  ob_convert12/1 -> ob_terminator12/1  "ob_OMAPve_y_ADAS_ACCStIconDis"
  ob_convert13/1 -> ob_terminator13/1  "ob_OMAPve_y_ADAS_ACC_RVVReqType"
  ob_convert14/1 -> ob_terminator14/1  "ob_OMAPve_y_ADAS_ACCMsgPrompt"
  ob_convert15/1 -> ob_terminator15/1  "ob_OMAPve_y_ADAS_AEBAlertReq"
  ob_convert16/1 -> ob_terminator16/1  "ob_OMAPve_y_ADAS_AEBFaultStatus"
  ob_convert17/1 -> ob_terminator17/1  "ob_OMAPve_y_ADAS_AEBSwitchSt"
  ob_convert18/1 -> ob_terminator18/1  "ob_OMAPve_y_ADAS_AEBMassageDisp"
  ob_convert19/1 -> ob_terminator19/1  "ob_OMAPve_y_ADAS_HMITargDispFlg"
  ob_convert20/1 -> ob_terminator20/1  "ob_OMAPve_y_ADAS_TargetPosition"
  ob_convert23/1 -> ob_terminator23/1  "ob_OMAPve_g_ADAS_ACCTorqueReq"
  ob_convert24/1 -> ob_terminator24/1  "ob_OMAPve_y_ADAS_TorqueActivReq"
  ob_convert25/1 -> ob_terminator25/1  "ob_OMAPve_g_ADAS_DownUpMinTime"
  ob_convert26/1 -> ob_terminator26/1  "ob_OMAPve_y_ADAS_UpDownGearCng"
  ob_convert27/1 -> ob_terminator27/1  "ob_OMAPve_y_ADAS_ACCState"
  ob_convert28/1 -> ob_terminator28/1  "ob_OMAPve_g_ADAS_DecelSet"
  ob_convert29/1 -> ob_terminator29/1  "ob_OMAPve_y_ADAS_DeclControlReq"
  ob_convert30/1 -> ob_terminator30/1  "ob_OMAPve_y_ADAS_PrefillRequest"
  ob_convert31/1 -> ob_terminator31/1  "ob_OMAPve_y_ADAS_ESCDriveOff"
  ob_convert32/1 -> ob_terminator32/1  "ob_OMAPve_y_ADAS_ESCHoldReq"
  ob_convert33/1 -> ob_terminator33/1  "ob_OMAPve_y_ADAS_DecelType"
  ob_convert34/1 -> ob_terminator34/1  "ob_OMAPve_y_ADAS_AEBState"
  ob_convert35/1 -> ob_terminator35/1  "ob_OMAPve_y_ADAS_BrakeRequest"
  ob_convert36/1 -> ob_terminator36/1  "ob_OMAPve_y_ADAS_AEBBrakingProg"
  ob_convert37/1 -> ob_terminator37/1  "ob_OMAPve_y_ADAS_HapticAlarmReq"
  ob_convert38/1 -> ob_terminator38/1  "ob_OMAPve_y_ADAS_Handsoffwarn"
  ob_convert39/1 -> ob_terminator39/1  "ob_OMAPve_y_ADAS_HMIPopupMsg"
  ob_convert40/1 -> ob_terminator40/1  "ob_OMAPve_y_ADAS_VehicleLaneDis"
  ob_convert41/1 -> ob_terminator41/1  "ob_OMAPve_y_ADAS_LDWWarningSt"
  ob_convert42/1 -> ob_terminator42/1  "ob_OMAPve_y_ADAS_LDWStatusDisp"
  ob_convert43/1 -> ob_terminator43/1  "ob_OMAPve_y_ADAS_LKAMode"
  ob_convert44/1 -> ob_terminator44/1  "ob_OMAPve_y_ADAS_LKAStatusDisp"
  ob_convert45/1 -> ob_terminator45/1  "ob_OMAPve_y_ADAS_LKASwitchState"
  ob_convert46/1 -> ob_terminator46/1  "ob_OMAPve_y_ADAS_ELKSts"
  ob_convert47/1 -> ob_terminator47/1  "ob_OMAPve_y_ADAS_LCAStatusDisp"
  ob_convert48/1 -> ob_terminator48/1  "ob_OMAPve_y_ADAS_LCAPopupMsg"
  ob_convert49/1 -> ob_terminator49/1  "ob_OMAPve_y_ADAS_LKAState"
  ob_convert50/1 -> ob_terminator50/1  "ob_OMAPve_g_ADAS_LKATorqFactReq"
  ob_convert51/1 -> ob_terminator51/1  "ob_OMAPve_g_ADAS_LKAAngleReq"
  ob_convert52/1 -> ob_terminator52/1  "ob_OMAPve_y_ADAS_LKAActivation"
  ob_convert53/1 -> ob_terminator53/1  "ob_OMAPve_y_ADAS_ESAState"
  ob_convert54/1 -> ob_terminator54/1  "ob_OMAPve_g_ADAS_ESATorqueReq"
  ob_convert55/1 -> ob_terminator55/1  "ob_OMAPve_y_ADAS_ESARequest"
  ob_convert56/1 -> ob_terminator56/1  "ob_OMAPve_y_ADAS_ICAMassageDisp"
  ob_convert57/1 -> ob_terminator57/1  "ob_OMAPve_y_ADAS_ICAStatusIcon"
  ob_convert58/1 -> ob_terminator58/1  "ob_OMAPve_y_ADAS_HWAMode"
  ob_convert59/1 -> ob_terminator59/1  "ob_OMAPve_y_ADAS_HWATurnOnIdctr"
  ob_convert60/1 -> ob_terminator60/1  "ob_OMAPve_y_ADAS_ESAFaultSt"
  ob_convert61/1 -> ob_terminator61/1  "ob_OMAPve_y_ADAS_JAFaultSt"
  ob_convert62/1 -> ob_terminator62/1  "ob_OMAPve_y_ADAS_HWAActionSts"
  ob_convert63/1 -> ob_terminator63/1  "ob_OMAPve_y_ADAS_OperatingSt"
  ob_convert66/1 -> ob_terminator66/1  "ob_OMAPve_y_ADAS_Radar_State"
  ob_convert67/1 -> ob_terminator67/1  "ob_OMAPve_y_ADAS_ACCRequestEPB"
  ob_convert70/1 -> ob_terminator70/1  "ob_OMAPve_y_ADAS_State"
  ob_convert72/1 -> ob_terminator72/1  "ob_OMAPve_y_ADAS_TrnLgtsCmd"
  ob_convert73/1 -> ob_terminator73/1  "ob_OMAPve_y_ADAS_LightCtrlValid"
  Subsystem6/7(Out7) -> OMAPve_y_ADAS_ISLCState/1, ob_convert6/1
  Subsystem6/8(Out8) -> OMAPve_y_ADAS_ISLCDriverRemind/1, ob_convert7/1
  Subsystem7/1(Out1) -> OMAPve_y_ADAS_LCAStatusDisplay/1, ob_convert47/1
  Subsystem7/2(Out2) -> OMAPve_y_ADAS_LCAPopupMessage/1, ob_convert48/1
  Subsystem4/5(Out5) -> ob_convert53/1, OMAPve_y_ADAS_ESAState/1
  Subsystem4/7(Out7) -> ob_convert55/1, OMAPve_y_ADAS_ESARequest/1
  Subsystem4/6(Out6) -> ob_convert54/1, OMAPve_g_ADAS_ESATorqueReq/1
  Subsystem6/3(Out3) -> ob_convert58/1, OMAPve_y_ADAS_HWAMode/1
  Subsystem6/4(Out4) -> ob_convert59/1, OMAPve_y_ADAS_HWATurnOnIdctr/1
  Subsystem6/2(Out2) -> ob_convert60/1, OMAPve_y_ADAS_ESAFaultSt/1
  Subsystem6/5(Out5) -> OMAPve_y_ADAS_HWAActionSts/1, ob_convert62/1
  Subsystem6/6(Out6) -> OMAPve_y_ADAS_LightControlValid/1, ob_convert73/1
  Subsystem7/3(Out3) -> OMAPve_y_ADAS_State/1, ob_convert70/1
  ICABve_g_LKATorqueReq_Value/1 -> Gain11/1
  ICABve_d_LKATorqueReq/1 -> Gain12/1
  Data Type Conversion84/1 -> Bus_ACCS/18  "ACCSve_d_ACC_GoIndicateReq_LZM_convert"
  Data Type Conversion109/1 -> Bus_LKAS/10  "LKASve_g_EPS_Factor_Control_convert"
  Data Type Conversion175/1 -> Bus_JABS/13  "JABSve_d_DbTips_convert"
  Data Type Conversion177/1 -> Bus_JABS/15  "JABSve_d_DbESCHoldReq_convert"
  Data Type Conversion173/1 -> Bus_JABS/11  "JABSve_d_DbFltStatus_convert"
  ELKSve_g_EPS_Factor_Control/1 -> Data Type Conversion145/1, ob_In_convert83/1
  IMAPve_g_ESC_LonAcc/1 -> Data Type Conversion56/1, ob_In_convert118/1
  Data Type Conversion140/1 -> Bus_ELKS/3  "ELKSve_y_Hands_Off_Warning_convert"
  Data Type Conversion92/1 -> Bus_ACCS/4  "ACCSve_g_ACC_DecReq_convert"
  Data Type Conversion116/1 -> Bus_LKAS/3  "LKASve_y_LKA_Status_Display_convert"
  Data Type Conversion170/1 -> Bus_JABS/7  "JABSve_d_DbBraking_progress_convert"
  Data Type Conversion93/1 -> Bus_ACCS/3  "ACCSve_d_ACC_TqFlag_convert"
  Data Type Conversion56/1 -> Bus_IMAP/2  "IMAPve_g_ESC_LonAcc_convert"
  ELKSve_y_ELK_HapticAlarmReq/1 -> Data Type Conversion139/1, ob_In_convert77/1
  Data Type Conversion171/1 -> Bus_JABS/9  "JABSve_d_DbJACWStatus_convert"
  Data Type Conversion141/1 -> Bus_ELKS/4  "ELKSve_y_ELK_Action_Indication_convert"
  JABSve_d_DbTips/1 -> Data Type Conversion175/1, ob_In_convert62/1
  ACCSve_d_VelocitySet/1 -> Data Type Conversion62/1, ob_In_convert21/1
  Data Type Conversion169/1 -> Bus_JABS/6  "JABSve_d_DbHapticAlarm_convert"
  Data Type Conversion82/1 -> Bus_ACCS/16  "ACCSve_d_ACC_CtlVeh_LZM_convert"
  Data Type Conversion2/1 -> Bus_ACCS/14  "ACCSve_d_ACC_ESCHoldReq_convert"
  Data Type Conversion165/1 -> Bus_JABS/2  "JABSve_d_DbFunFARCSta_convert"
  JABSve_d_DbHapticAlarm/1 -> Data Type Conversion169/1, ob_In_convert55/1
  Data Type Conversion161/1 -> Bus_AEBS/3  "AEBSve_g_DecSetpoint_convert"
  FDMMve_d_SignalTStamp/1 -> Data Type Conversion21/1, ob_In_convert12/1
  Ground2/1 -> Data Type Conversion27/1, ob_In_convert94/1
  Data Type Conversion147/1 -> Bus_ELKS/10  "ELKSve_y_ELK_VehicleLaneDisp_convert"
  Data Type Conversion158/1 -> Bus_AEBS/6  "AEBSve_d_ESCDriveOff_convert"
  Data Type Conversion58/1 -> Bus_FDMM/4  "FDMMve_d_ElkFcnConf_convert"
  AEBSve_d_JABS_FltStatus/1 -> Data Type Conversion6/1, ob_In_convert46/1
  Data Type Conversion154/1 -> Bus_AEBS/10  "AEBSve_d_AEBStatus_convert"
  Data Type Conversion150/1 -> Bus_AEBS/14  "AEBSve_d_AEBAlertReq_convert"
  Data Type Conversion145/1 -> Bus_ELKS/8  "ELKSve_g_EPS_Factor_Control_convert"
  IMAPve_g_R0_C0/1 -> Data Type Conversion105/1, ob_In_convert126/1
  Data Type Conversion163/1 -> Bus_AEBS/1  "AEBSve_d_Prefill_request_convert"
  LKASve_y_LKATorqueReq/1 -> Gain8/1
  Data Type Conversion160/1 -> Bus_AEBS/4  "AEBSve_d_MDDdecRequest_convert"
  Data Type Conversion95/1 -> Bus_ACCS/1  "ACCSve_d_ACC_State_convert"
  JABSve_d_DbFunFARCSta/1 -> Data Type Conversion165/1, ob_In_convert51/1
  ELKSve_y_EPS_ELK_Control/1 -> Data Type Conversion146/1, ob_In_convert84/1
  Data Type Conversion162/1 -> Bus_AEBS/2  "AEBSve_d_functionFARCState_convert"
  Data Type Conversion155/1 -> Bus_AEBS/9  "AEBSve_d_Braking_progress_convert"
  AEBSve_d_AEBSwitchStatus/1 -> Data Type Conversion152/1, ob_In_convert39/1
  Data Type Conversion79/1 -> Bus_AEBS/24  "AEBSve_d_DAS1_Status_DBS_Enable_convert"
  Data Type Conversion21/1 -> Bus_FDMM/12  "FDMMve_d_SignalTStamp_convert"
  ACCSve_d_ACC_ESCHoldReq/1 -> ob_In_convert26/1, Data Type Conversion2/1
  AEBSve_d_JABS_HapticAlarm/1 -> Data Type Conversion5/1, ob_In_convert48/1
  JABSve_d_DbJACWStatus/1 -> Data Type Conversion171/1, ob_In_convert58/1
  Ground8/1 -> ob_In_convert136/1, Data Type Conversion79/1
  Data Type Conversion182/1 -> Bus_ICA/8  "ICABve_g_LKATorqueReq_Value_convert"
  Data Type Conversion148/1 -> Bus_ELKS/11  "ELKSve_y_ELK_ELKSts_convert"
  IMAPve_d_ESC_Veh_Standstill/1 -> Data Type Conversion100/1, ob_In_convert121/1
  JABSve_d_DbSignalTStamp/1 -> Data Type Conversion30/1, ob_In_convert57/1
  Data Type Conversion178/1 -> Bus_ELKS/13  "ELKSve_y_LKATorqueReq_convert"
  Data Type Conversion151/1 -> Bus_AEBS/13  "AEBSve_d_AEBFaultStatus_convert"
  Ground11/1 -> ob_In_convert131/1, Data Type Conversion83/1
  Ground13/1 -> ob_In_convert133/1, Data Type Conversion85/1
  ACCSve_d_ACC_go_request/1 -> ob_In_convert20/1, Data Type Conversion63/1
  ACCSve_d_SignalTStamp/1 -> ob_In_convert23/1, Data Type Conversion3/1
  AEBSve_d_ESCDriveOff/1 -> Data Type Conversion158/1, ob_In_convert33/1
  ACCSve_d_ACC_EPBReq/1 -> ob_In_convert27/1, Data Type Conversion/1
  LKASve_y_LKA_Status_Display/1 -> Data Type Conversion116/1, ob_In_convert67/1
  Data Type Conversion180/1 -> Bus_ICA/7  "ICABve_d_LKATorqueReq_convert"
  JABSve_d_DbPrefillReq/1 -> Data Type Conversion164/1, ob_In_convert50/1
  LKASve_g_LKA_SWA_Control/1 -> Data Type Conversion110/1, ob_In_convert73/1
  Data Type Conversion23/1 -> Bus_ICA/1  "ICABva_d_PathQI_convert"
  AEBSve_d_AEBAlertReq/1 -> Data Type Conversion150/1, ob_In_convert41/1
  Data Type Conversion15/1 -> Bus_FDMM/9  "FDMMve_d_AlcFcnConf_convert"
  ACCSve_d_ACC_ESCDriveOff/1 -> ob_In_convert25/1, Data Type Conversion1/1
  Data Type Conversion172/1 -> Bus_JABS/10  "JABSve_d_DbSwitchStatus_convert"
  JABSve_d_DbAlertReq/1 -> Data Type Conversion174/1, ob_In_convert61/1
  Ground14/1 -> ob_In_convert134/1, Data Type Conversion86/1
  Data Type Conversion27/1 -> Bus_ICA/9  "ICADva_d_DecionState_convert"
  Ground3/1 -> Data Type Conversion26/1, ob_In_convert95/1
  IMAPve_g_R0_C2/1 -> Data Type Conversion107/1, ob_In_convert128/1
  Ground7/1 -> ob_In_convert137/1, Data Type Conversion80/1
  Data Type Conversion112/1 -> Bus_LKAS/7  "LKASve_y_HMI_Popup_Status_convert"
  LKASve_y_EPS_LKA_Control/1 -> Data Type Conversion119/1, ob_In_convert75/1
  ELKSve_y_LKATorqueReq/1 -> Gain10/1
  Ground12/1 -> ob_In_convert132/1, Data Type Conversion84/1
  Data Type Conversion89/1 -> Bus_ACCS/7  "ACCSve_d_ACCActive_Signal_convert"
  Data Type Conversion102/1 -> Bus_IMAP/7  "IMAPve_g_L0_C1_convert"
  Data Type Conversion157/1 -> Bus_AEBS/7  "AEBSve_d_ESCHoldReq_convert"
  ELKSve_g_ELK_SWA_Control/1 -> Data Type Conversion144/1, ob_In_convert82/1
  Data Type Conversion98/1 -> Bus_IMAP/3  "IMAPva_d_obj_id_convert"
  Data Type Conversion91/1 -> Bus_ACCS/5  "ACCSve_d_ACC_DecFlag_convert"
  AEBSve_d_HapticAlarm/1 -> Data Type Conversion156/1, ob_In_convert35/1
  Data Type Conversion96/1 -> Bus_ACCS/12  "ACCSve_d_ACC_ICA_Flag_convert"
  Data Type Conversion62/1 -> Bus_ACCS/9  "ACCSve_d_VelocitySet_convert"
  Data Type Conversion20/1 -> Bus_FDMM/8  "FDMMve_d_LfFcnConf_convert"
  ICABve_d_ICAState/1 -> Data Type Conversion24/1, ob_In_convert93/1
  Data Type Conversion54/1 -> Bus_ICA/4  "ICABve_g_SteerAngleCmd_convert"
  ELKSve_y_SignalTStamp/1 -> Data Type Conversion11/1, ob_In_convert87/1
  Data Type Conversion57/1 -> Bus_FDMM/5  "FDMMve_d_LkaFcnConf_convert"
  Data Type Conversion83/1 -> Bus_ACCS/17  "ACCSve_d_ACC_CancelReq_LZM_convert"
  Data Type Conversion85/1 -> Bus_ACCS/19  "ACCSve_d_ACC_OverrideIndReq_LZM_convert"
  Data Type Conversion86/1 -> Bus_ACCS/20  "AACCSve_d_ACC_TakeoverIndReq_LZM_convert"
  IMAPve_d_EPS_LKA_State/1 -> Data Type Conversion97/1, ob_In_convert117/1
  FDMMve_g_Adas2Fapa/1 -> Data Type Conversion22/1, ob_In_convert11/1
  AEBSve_d_AEBTips/1 -> Data Type Conversion149/1, ob_In_convert42/1
  Data Type Conversion87/1 -> Bus_LKAS/12  "LKASve_y_LKATorqueReq_convert"
  Data Type Conversion179/1 -> Bus_ELKS/14  "ELKSve_g_LKATorqueReq_Value_convert"
  Ground/1 -> Data Type Conversion20/1, ob_In_convert8/1
  LKASve_g_LKATorqueReq_Value/1 -> Gain7/1
  Data Type Conversion78/1 -> Bus_AEBS/23  "AEBSve_d_DAS1_Status_AEBJerkWarning_Lvl_convert"
  AEBSve_d_Prefill_request/1 -> Data Type Conversion163/1, ob_In_convert28/1
  ELKSve_y_Hands_Off_Warning/1 -> Data Type Conversion140/1, ob_In_convert78/1
  ELKSve_y_EPS_State_Control/1 -> Data Type Conversion143/1, ob_In_convert81/1
  AEBSve_d_Braking_progress/1 -> Data Type Conversion155/1, ob_In_convert36/1
  Data Type Conversion168/1 -> Bus_JABS/5  "JABSve_d_DbMDDdecType_convert"
  ACCSve_g_ACC_TqReq/1 -> ob_In_convert14/1, Data Type Conversion94/1
  ICABve_d_SignalTStamp/1 -> Data Type Conversion25/1, ob_In_convert89/1
  AEBSve_d_JABS_AlertSign/1 -> Data Type Conversion7/1, ob_In_convert44/1
  Bus_ACCS/1 -> ACCS_Direct/1(Input_ACCS)  "Input_ACCS"
  IMAPve_g_L0_C3/1 -> Data Type Conversion104/1, ob_In_convert125/1
  ELKSve_y_ELK_Action_Indication/1 -> Data Type Conversion141/1, ob_In_convert79/1
  ICABve_d_ICAMode/1 -> Data Type Conversion55/1, ob_In_convert92/1
  Data Type Conversion28/1 -> Bus_ICA/11  "ICADva_d_LCRecommend_convert"
  ELKSve_y_HMI_Popup_Status/1 -> Data Type Conversion142/1, ob_In_convert80/1
  Data Type Conversion11/1 -> Bus_ELKS/12  "ELKSve_y_SignalTStamp_convert"
  IMAPve_g_R0_C3/1 -> Data Type Conversion108/1, ob_In_convert129/1
  FDMMve_d_ElkFcnConf/1 -> Data Type Conversion58/1, ob_In_convert4/1
  LKASve_y_EPS_State_Control/1 -> Data Type Conversion111/1, ob_In_convert72/1
  LKASve_y_HMI_Popup_Status/1 -> Data Type Conversion112/1, ob_In_convert71/1
  Data Type Conversion55/1 -> Bus_ICA/5  "ICABve_d_ICAMode_convert"
  FDMMve_d_JaFcnConf/1 -> Data Type Conversion19/1, ob_In_convert1/1
  AEBSve_d_functionFARCState/1 -> Data Type Conversion162/1, ob_In_convert29/1
  IMAPva_g_obj_pos_x/1 -> Data Type Conversion99/1, ob_In_convert120/1
  FDMMve_d_EwFcnConf/1 -> Data Type Conversion17/1, ob_In_convert10/1
  IMAPve_g_L0_C0/1 -> Data Type Conversion101/1, ob_In_convert122/1
  JABSve_d_DbBraking_progress/1 -> Data Type Conversion170/1, ob_In_convert56/1
  Data Type Conversion16/1 -> Bus_FDMM/3  "FDMMve_d_EsaFcnConf_convert"
  ACCSve_d_ACC_DecFlag/1 -> ob_In_convert17/1, Data Type Conversion91/1
  AEBSve_d_ESCHoldReq/1 -> Data Type Conversion157/1, ob_In_convert34/1
  Data Type Conversion26/1 -> Bus_ICA/10  "ICADva_d_DecionCMD_convert"
  Data Type Conversion99/1 -> Bus_IMAP/4  "IMAPva_g_obj_pos_x_convert"
  Data Type Conversion149/1 -> Bus_AEBS/15  "AEBSve_d_AEBTips_convert"
  ELKSve_y_state_ELK_function/1 -> Data Type Conversion12/1, ob_In_convert76/1
  LKASve_y_LKA_Action_Indication/1 -> Data Type Conversion113/1, ob_In_convert70/1
  ACCSve_d_ACC_ICA_Flag/1 -> ob_In_convert24/1, Data Type Conversion96/1
  Data Type Conversion22/1 -> Bus_FDMM/11  "FDMMve_g_Adas2Fapa_convert"
  FDMMve_d_EsaFcnConf/1 -> Data Type Conversion16/1, ob_In_convert3/1
  Data Type Conversion6/1 -> Bus_AEBS/19  "AEBSve_d_JABS_FltStatus_convert"
  Data Type Conversion174/1 -> Bus_JABS/12  "JABSve_d_DbAlertReq_convert"
  ACCSve_d_ACCActive_Signal/1 -> ob_In_convert19/1, Data Type Conversion89/1
  Data Type Conversion159/1 -> Bus_AEBS/5  "AEBSve_d_MDDdecType_convert"
  Data Type Conversion9/1 -> Bus_AEBS/22  "AEBSve_d_JABS_Tips_convert"
  AEBSve_g_DecSetpoint/1 -> Data Type Conversion161/1, ob_In_convert30/1
  FDMMve_d_AccFcnConf/1 -> Data Type Conversion13/1, ob_In_convert7/1
  Ground5/1 -> Data Type Conversion29/1, ob_In_convert97/1
  ACCSve_d_CIPV_ID/1 -> ob_In_convert18/1, Data Type Conversion90/1
  FDMMve_d_LkaFcnConf/1 -> Data Type Conversion57/1, ob_In_convert5/1
  JABSve_d_DbESCHoldReq/1 -> Data Type Conversion177/1, ob_In_convert64/1
  IMAPve_g_L0_C1/1 -> Data Type Conversion102/1, ob_In_convert123/1
  Data Type Conversion/1 -> Bus_ACCS/15  "ACCSve_d_ACC_EPBReq_convert"
  Data Type Conversion13/1 -> Bus_FDMM/7  "FDMMve_d_AccFcnConf_convert"
  Data Type Conversion17/1 -> Bus_FDMM/10  "FDMMve_d_EwFcnConf_convert"
  FDMMve_d_IcaFcnConf/1 -> Data Type Conversion18/1, ob_In_convert6/1
  Data Type Conversion24/1 -> Bus_ICA/6  "ICABve_d_ICAState_convert"
  Data Type Conversion25/1 -> Bus_ICA/2  "ICABve_d_SignalTStamp_convert"
  Data Type Conversion18/1 -> Bus_FDMM/6  "FDMMve_d_IcaFcnConf_convert"
  AEBSve_d_JABS_Tips/1 -> Data Type Conversion9/1, ob_In_convert49/1
  Data Type Conversion4/1 -> Bus_AEBS/20  "AEBSve_d_JABS_AlertReq_convert"
  LKASve_g_EPS_Factor_Control/1 -> Data Type Conversion109/1, ob_In_convert74/1
  ACCSve_d_HeadWaySet/1 -> ob_In_convert22/1, Data Type Conversion60/1
  AEBSve_d_AEBStatus/1 -> Data Type Conversion154/1, ob_In_convert37/1
  Data Type Conversion60/1 -> Bus_ACCS/10  "ACCSve_d_HeadWaySet_convert"
  Data Type Conversion146/1 -> Bus_ELKS/9  "ELKSve_y_EPS_ELK_Control_convert"
  Data Type Conversion139/1 -> Bus_ELKS/2  "ELKSve_y_ELK_HapticAlarmReq_convert"
  Data Type Conversion90/1 -> Bus_ACCS/6  "ACCSve_d_CIPV_ID_convert"
  Data Type Conversion166/1 -> Bus_JABS/3  "JABSve_g_DbDecSetpoint_convert"
  ACCSve_d_ACC_TqFlag/1 -> ob_In_convert15/1, Data Type Conversion93/1
  ACCSve_d_ACC_State/1 -> ob_In_convert13/1, Data Type Conversion95/1
  Data Type Conversion153/1 -> Bus_AEBS/11  "AEBSve_d_FCWStatus_convert"
  Data Type Conversion105/1 -> Bus_IMAP/10  "IMAPve_g_R0_C0_convert"
  Data Type Conversion30/1 -> Bus_JABS/8  "JABSve_d_DbSignalTStamp_convert"
  Data Type Conversion118/1 -> Bus_LKAS/1  "LKASve_y_Vehicle_Lane_Display_convert"
  Data Type Conversion101/1 -> Bus_IMAP/6  "IMAPve_g_L0_C0_convert"
  LKASve_y_LDW_Status_Display/1 -> Data Type Conversion117/1, ob_In_convert66/1
  ACCSve_g_ACC_DecReq/1 -> ob_In_convert16/1, Data Type Conversion92/1
  Data Type Conversion142/1 -> Bus_ELKS/5  "ELKSve_y_HMI_Popup_Status_convert"
  Data Type Conversion97/1 -> Bus_IMAP/1  "IMAPve_d_EPS_LKA_State_convert"
  Data Type Conversion119/1 -> Bus_LKAS/11  "LKASve_y_EPS_LKA_Control_convert"
  Data Type Conversion100/1 -> Bus_IMAP/5  "IMAPve_d_ESC_Veh_Standstill_convert"
  Data Type Conversion117/1 -> Bus_LKAS/2  "LKASve_y_LDW_Status_Display_convert"
  LKASve_y_Hands_Off_Warning/1 -> Data Type Conversion114/1, ob_In_convert69/1
  Data Type Conversion115/1 -> Bus_LKAS/4  "LKASve_y_LDW_Flag_convert"
  Data Type Conversion19/1 -> Bus_FDMM/1  "FDMMve_d_JaFcnConf_convert"
  JABSve_d_DbMDDdecType/1 -> Data Type Conversion168/1, ob_In_convert54/1
  Data Type Conversion111/1 -> Bus_LKAS/8  "LKASve_y_EPS_State_Control_convert"
  AEBSve_d_JABS_SwitchStatus/1 -> Data Type Conversion8/1, ob_In_convert45/1
  Data Type Conversion7/1 -> Bus_AEBS/17  "AEBSve_d_JABS_AlertSign_convert"
  Data Type Conversion107/1 -> Bus_IMAP/12  "IMAPve_g_R0_C2_convert"
  Data Type Conversion167/1 -> Bus_JABS/4  "JABSve_d_DbMDDdecRequest_convert"
  Data Type Conversion88/1 -> Bus_LKAS/13  "LKASve_g_LKATorqueReq_Value_convert"
  Data Type Conversion29/1 -> Bus_ICA/12  "ICADve_d_SignalTStamp_convert"
  AEBSve_d_FCWStatus/1 -> Data Type Conversion153/1, ob_In_convert38/1
  Ground6/1 -> ob_In_convert138/1, Data Type Conversion81/1
  AEBSve_d_SignalTStamp/1 -> Data Type Conversion10/1, ob_In_convert43/1
  Data Type Conversion176/1 -> Bus_JABS/14  "JABSve_d_DbESCDriveOff_convert"
  ELKSve_y_ELK_VehicleLaneDisp/1 -> Data Type Conversion147/1, ob_In_convert85/1
  AEBSve_d_JABS_AlertReq/1 -> Data Type Conversion4/1, ob_In_convert47/1
  Data Type Conversion14/1 -> Bus_FDMM/2  "FDMMve_d_AebFcnConf_convert"
  JABSve_d_DbMDDdecRequest/1 -> Data Type Conversion167/1, ob_In_convert53/1
  IMAPva_d_obj_id/1 -> Data Type Conversion98/1, ob_In_convert119/1
  IMAPve_g_R0_C1/1 -> Data Type Conversion106/1, ob_In_convert127/1
  AEBSve_d_MDDdecType/1 -> Data Type Conversion159/1, ob_In_convert32/1
  Data Type Conversion10/1 -> Bus_AEBS/16  "AEBSve_d_SignalTStamp_convert"
  ELKSve_g_LKATorqueReq_Value/1 -> Gain9/1
  Data Type Conversion113/1 -> Bus_LKAS/6  "LKASve_y_LKA_Action_Indication_convert"
  Data Type Conversion110/1 -> Bus_LKAS/9  "LKASve_g_LKA_SWA_Control_convert"
  JABSve_g_DbDecSetpoint/1 -> Data Type Conversion166/1, ob_In_convert52/1
  Data Type Conversion156/1 -> Bus_AEBS/8  "AEBSve_d_HapticAlarm_convert"
  Data Type Conversion1/1 -> Bus_ACCS/13  "ACCSve_d_ACC_ESCDriveOff_convert"
  JABSve_d_DbSwitchStatus/1 -> Data Type Conversion172/1, ob_In_convert59/1
  FDMMve_d_AebFcnConf/1 -> Data Type Conversion14/1, ob_In_convert2/1
  AEBSve_d_MDDdecRequest/1 -> Data Type Conversion160/1, ob_In_convert31/1
  Data Type Conversion144/1 -> Bus_ELKS/7  "ELKSve_g_ELK_SWA_Control_convert"
  ICABve_g_SteerAngleCmd/1 -> Data Type Conversion54/1, ob_In_convert91/1
  Ground4/1 -> Data Type Conversion28/1, ob_In_convert96/1
  IMAPve_g_L0_C2/1 -> Data Type Conversion103/1, ob_In_convert124/1
  Bus Creator/1 -> ESAS_Direct/1(Input_ESAS), [ESA_Input]  "Input_ESAS"
  ? -> Data Type Conversion23/1, ob_In_convert88/1
  Ground1/1 -> Data Type Conversion15/1, ob_In_convert9/1
  JABSve_d_DbESCDriveOff/1 -> Data Type Conversion176/1, ob_In_convert63/1
  AEBSve_d_AEBFaultStatus/1 -> Data Type Conversion151/1, ob_In_convert40/1
  Data Type Conversion103/1 -> Bus_IMAP/8  "IMAPve_g_L0_C2_convert"
  ELKSve_y_ELK_ELKSts/1 -> Data Type Conversion148/1, ob_In_convert86/1
  Data Type Conversion8/1 -> Bus_AEBS/18  "AEBSve_d_JABS_SwitchStatus_convert"
  Data Type Conversion63/1 -> Bus_ACCS/8  "ACCSve_d_ACC_go_request_convert"
  Data Type Conversion143/1 -> Bus_ELKS/6  "ELKSve_y_EPS_State_Control_convert"
  LKASve_y_LDW_Flag/1 -> Data Type Conversion115/1, ob_In_convert68/1
  Data Type Conversion114/1 -> Bus_LKAS/5  "LKASve_y_Hands_Off_Warning_convert"
  Data Type Conversion3/1 -> Bus_ACCS/11  "ACCSve_d_SignalTStamp_convert"
  Bus_FDMM/1 -> [FD_Input]  "Input_FDMM"
  Data Type Conversion108/1 -> Bus_IMAP/13  "IMAPve_g_R0_C3_convert"
  Data Type Conversion152/1 -> Bus_AEBS/12  "AEBSve_d_AEBSwitchStatus_convert"
  Bus_JABS/1 -> JABS_Direct/1(Input_JABS)  "Input_JABS"
  Bus_ELKS/1 -> ELKS_Direct/1(Input_ELKS)  "Input_ELKS"
  LKASve_y_Vehicle_Lane_Display/1 -> Data Type Conversion118/1, ob_In_convert65/1
  JABSve_d_DbFltStatus/1 -> Data Type Conversion173/1, ob_In_convert60/1
  ICABva_d_ICAB2HMI/1 -> Data Type Conversion31/1, ob_In_convert90/1
  Data Type Conversion31/1 -> Bus_ICA/3  "ICABva_d_ICAB2HMI_convert"
  Data Type Conversion80/1 -> Bus_AEBS/25  "AEBSve_d_DAS1_Status_FCW_DBSReq_convert"
  ESASve_y_ESA_State/1 -> Data Type Conversion42/1, Data Type Conversion33/1
  Data Type Conversion104/1 -> Bus_IMAP/9  "IMAPve_g_L0_C3_convert"
  Data Type Conversion5/1 -> Bus_AEBS/21  "AEBSve_d_JABS_HapticAlarm_convert"
  Data Type Conversion12/1 -> Bus_ELKS/1  "ELKSve_y_state_ELK_function_convert"
  Data Type Conversion81/1 -> Bus_AEBS/26  "AEBSve_d_DAS3_Status_FCWWarning_Lvl_convert"
  Data Type Conversion94/1 -> Bus_ACCS/2  "ACCSve_g_ACC_TqReq_convert"
  Data Type Conversion106/1 -> Bus_IMAP/11  "IMAPve_g_R0_C1_convert"
  Bus_AEBS/1 -> AEBS_Direct/1(Input_AEBS)  "Input_AEBS"
  [FD_Input] -> AEBS_Direct/2(Input_FDMM)
  Bus_ICA/1 -> ICA_Direct_G59/1(Input_ICA)  "Input_ICA"
  [FD_Input] -> JABS_Direct/2(Input_FDMM)
  Ground9/1 -> ob_In_convert135/1, Data Type Conversion78/1
  Bus_IMAP/1 -> [IMAP_Input]
  Data Type Conversion164/1 -> Bus_JABS/1  "JABSve_d_DbPrefillReq_convert"
  Bus_LKAS/1 -> LKAS_Direct/1(Input_LKAS)  "Input_LKAS"
  [FD_Input] -> ACCS_Direct/2(Input_FDMM)
  [IMAP_Input] -> ACCS_Direct/3(Input_IMAP)
  [FD_Input] -> ICA_Direct_G59/2(Input_FDMM)
  [IMAP_Input] -> ICA_Direct_G59/3(Input_IMAP)
  [ACC_to_ICA] -> ICA_Direct_G59/4(ACC_to_ICA)
  Ground10/1 -> ob_In_convert130/1, Data Type Conversion82/1
  ob_In_convert130/1 -> ob_In_terminator130/1  "ob_OACC_ACC_CtlVeh_LZM"
  ob_In_convert131/1 -> ob_In_terminator131/1  "ob_OACC_ACC_CancelReq_LZM"
  ob_In_convert132/1 -> ob_In_terminator132/1  "ob_OACC_ACC_GoIndicateReq_LZM"
  ob_In_convert133/1 -> ob_In_terminator133/1  "ob_OACC_ACC_OverrideIndReq_LZM"
  ob_In_convert134/1 -> ob_In_terminator134/1  "ob_OACC_ACC_TakeoverIndReq_LZM"
  ob_In_convert135/1 -> ob_In_terminator135/1  "ob_OAEB_DAS1_AEBWarning"
  ob_In_convert136/1 -> ob_In_terminator136/1  "ob_OAEB_DAS1_DBS_Enable"
  ob_In_convert137/1 -> ob_In_terminator137/1  "ob_OAEB_DAS1_FCW_DBSReq"
  ob_In_convert138/1 -> ob_In_terminator138/1  "ob_OAEB_DAS3_FCWWarning"
  ob_In_convert139/1 -> ob_In_terminator139/1  "ob_OLKA_LKATorqueReq"
  ob_In_convert140/1 -> ob_In_terminator140/1  "ob_OLKA_LKATorqueReq_Value"
  ob_In_convert141/1 -> ob_In_terminator141/1  "ob_OELK_LKATorqueReq"
  ob_In_convert142/1 -> ob_In_terminator142/1  "ob_OELK_LKATorqueReq_Value"
  ob_In_convert143/1 -> ob_In_terminator143/1  "ob_OICAB_LKATorqueReq"
  ob_In_convert144/1 -> ob_In_terminator144/1  "ob_OICAB_LKATorqueReq_Value"
  ob_In_convert1/1 -> ob_In_terminator1/1  "ob_OFD_JaFcnConf"
  ob_In_convert2/1 -> ob_In_terminator2/1  "ob_OFD_AebFcnConf"
  ob_In_convert3/1 -> ob_In_terminator3/1  "ob_OFD_EsaFcnConf"
  ob_In_convert4/1 -> ob_In_terminator4/1  "ob_OFD_ElkFcnConf"
  ob_In_convert5/1 -> ob_In_terminator5/1  "ob_OFD_LkaFcnConf"
  ob_In_convert6/1 -> ob_In_terminator6/1  "ob_OFD_IcaFcnConf"
  ob_In_convert7/1 -> ob_In_terminator7/1  "ob_OFD_AccFcnConf"
  ob_In_convert8/1 -> ob_In_terminator8/1  "ob_OFD_LfFcnConf"
  ob_In_convert9/1 -> ob_In_terminator9/1  "ob_OFD_AlcFcnConf"
  ob_In_convert10/1 -> ob_In_terminator10/1  "ob_OFD_EwFcnConf"
  ob_In_convert11/1 -> ob_In_terminator11/1  "ob_OFD_Adas2Fapa"
  ob_In_convert12/1 -> ob_In_terminator12/1  "ob_OFD_SignalTStamp"
  ob_In_convert13/1 -> ob_In_terminator13/1  "ob_OACC_ACC_State"
  ob_In_convert14/1 -> ob_In_terminator14/1  "ob_OACC_ACC_TqReq"
  ob_In_convert15/1 -> ob_In_terminator15/1  "ob_OACC_ACC_TqFlag"
  ob_In_convert16/1 -> ob_In_terminator16/1  "ob_OACC_ACC_DecReq"
  ob_In_convert17/1 -> ob_In_terminator17/1  "ob_OACC_ACC_DecFlag"
  ob_In_convert18/1 -> ob_In_terminator18/1  "ob_OACC_CIPV_ID"
  ob_In_convert19/1 -> ob_In_terminator19/1  "ob_OACC_ACCActive_Signal"
  ob_In_convert20/1 -> ob_In_terminator20/1  "ob_OACC_ACC_go_request"
  ob_In_convert21/1 -> ob_In_terminator21/1  "ob_OACC_VelocitySet"
  ob_In_convert22/1 -> ob_In_terminator22/1  "ob_OACC_HeadWaySet"
  ob_In_convert23/1 -> ob_In_terminator23/1  "ob_OACC_SignalTStamp"
  ob_In_convert24/1 -> ob_In_terminator24/1  "ob_OACC_ACC_ICA_Flag"
  ob_In_convert25/1 -> ob_In_terminator25/1  "ob_OACC_ACC_ESCDriveOff"
  ob_In_convert26/1 -> ob_In_terminator26/1  "ob_OACC_ACC_ESCHoldReq"
  ob_In_convert27/1 -> ob_In_terminator27/1  "ob_OACC_ACC_EPBReq"
  ob_In_convert28/1 -> ob_In_terminator28/1  "ob_OAEB_Prefill_request"
  ob_In_convert29/1 -> ob_In_terminator29/1  "ob_OAEB_functionFARCState"
  ob_In_convert30/1 -> ob_In_terminator30/1  "ob_OAEB_DecSetpoint"
  ob_In_convert31/1 -> ob_In_terminator31/1  "ob_OAEB_MDDdecRequest"
  ob_In_convert32/1 -> ob_In_terminator32/1  "ob_OAEB_MDDdecType"
  ob_In_convert33/1 -> ob_In_terminator33/1  "ob_OAEB_ESCDriveOff"
  ob_In_convert34/1 -> ob_In_terminator34/1  "ob_OAEB_ESCHoldReq"
  ob_In_convert35/1 -> ob_In_terminator35/1  "ob_OAEB_HapticAlarm"
  ob_In_convert36/1 -> ob_In_terminator36/1  "ob_OAEB_Braking_progress"
  ob_In_convert37/1 -> ob_In_terminator37/1  "ob_OAEB_AEBStatus"
  ob_In_convert38/1 -> ob_In_terminator38/1  "ob_OAEB_FCWStatus"
  ob_In_convert39/1 -> ob_In_terminator39/1  "ob_OAEB_AEBSwitchStatus"
  ob_In_convert40/1 -> ob_In_terminator40/1  "ob_OAEB_AEBFaultStatus"
  ob_In_convert41/1 -> ob_In_terminator41/1  "ob_OAEB_AEBAlertReq"
  ob_In_convert42/1 -> ob_In_terminator42/1  "ob_OAEB_AEBTips"
  ob_In_convert43/1 -> ob_In_terminator43/1  "ob_OAEB_SignalTStamp"
  ob_In_convert44/1 -> ob_In_terminator44/1  "ob_OAEB_JABS_AlertSign"
  ob_In_convert45/1 -> ob_In_terminator45/1  "ob_OAEB_JABS_SwitchStatus"
  ob_In_convert46/1 -> ob_In_terminator46/1  "ob_OAEB_JABS_FltStatus"
  ob_In_convert47/1 -> ob_In_terminator47/1  "ob_OAEB_JABS_AlertReq"
  ob_In_convert48/1 -> ob_In_terminator48/1  "ob_OAEB_JABS_HapticAlarm"
  ob_In_convert49/1 -> ob_In_terminator49/1  "ob_OAEB_JABS_Tips"
  ob_In_convert50/1 -> ob_In_terminator50/1  "ob_OJAB_DbPrefillReq"
  ob_In_convert51/1 -> ob_In_terminator51/1  "ob_OJAB_DbFunFARCSta"
  ob_In_convert52/1 -> ob_In_terminator52/1  "ob_OJAB_DbDecSetpoint"
  ob_In_convert53/1 -> ob_In_terminator53/1  "ob_OJAB_DbMDDdecRequest"
  ob_In_convert54/1 -> ob_In_terminator54/1  "ob_OJAB_DbMDDdecType"
  ob_In_convert55/1 -> ob_In_terminator55/1  "ob_OJAB_DbHapticAlarm"
  ob_In_convert56/1 -> ob_In_terminator56/1  "ob_OJAB_DbBraking_progress"
  ob_In_convert57/1 -> ob_In_terminator57/1  "ob_OJAB_DbSignalTStamp"
  ob_In_convert58/1 -> ob_In_terminator58/1  "ob_OJAB_DbJACWStatus"
  ob_In_convert59/1 -> ob_In_terminator59/1  "ob_OJAB_DbSwitchStatus"
  ob_In_convert60/1 -> ob_In_terminator60/1  "ob_OJAB_DbFltStatus"
  ob_In_convert61/1 -> ob_In_terminator61/1  "ob_OJAB_DbAlertReq"
  ob_In_convert62/1 -> ob_In_terminator62/1  "ob_OJAB_DbTips"
  ob_In_convert63/1 -> ob_In_terminator63/1  "ob_OJAB_DbESCDriveOff"
  ob_In_convert64/1 -> ob_In_terminator64/1  "ob_OJAB_DbESCHoldReq"
  ob_In_convert65/1 -> ob_In_terminator65/1  "ob_OLKA_Vehicle_Lane_Display"
  ob_In_convert66/1 -> ob_In_terminator66/1  "ob_OLKA_LDW_Status_Display"
  ob_In_convert67/1 -> ob_In_terminator67/1  "ob_OLKA_LKA_Status_Display"
  ob_In_convert68/1 -> ob_In_terminator68/1  "ob_OLKA_LDW_Flag"
  ob_In_convert69/1 -> ob_In_terminator69/1  "ob_OLKA_Hands_Off_Warning"
  ob_In_convert70/1 -> ob_In_terminator70/1  "ob_OLKA_LKA_Action_Indication"
  ob_In_convert71/1 -> ob_In_terminator71/1  "ob_OLKA_HMI_Popup_Status"
  ob_In_convert72/1 -> ob_In_terminator72/1  "ob_OLKA_EPS_State_Control"
  ob_In_convert73/1 -> ob_In_terminator73/1  "ob_OLKA_LKA_SWA_Control"
  ob_In_convert74/1 -> ob_In_terminator74/1  "ob_OLKA_EPS_Factor_Control"
  ob_In_convert75/1 -> ob_In_terminator75/1  "ob_OLKA_EPS_LKA_Control"
  ob_In_convert76/1 -> ob_In_terminator76/1  "ob_OELK_state_ELK_function"
  ob_In_convert77/1 -> ob_In_terminator77/1  "ob_OELK_ELK_HapticAlarmReq"
  ob_In_convert78/1 -> ob_In_terminator78/1  "ob_OELK_Hands_Off_Warning"
  ob_In_convert79/1 -> ob_In_terminator79/1  "ob_OELK_ELK_Action_Indication"
  ob_In_convert80/1 -> ob_In_terminator80/1  "ob_OELK_HMI_Popup_Status"
  ob_In_convert81/1 -> ob_In_terminator81/1  "ob_OELK_EPS_State_Control"
  ob_In_convert82/1 -> ob_In_terminator82/1  "ob_OELK_ELK_SWA_Control"
  ob_In_convert83/1 -> ob_In_terminator83/1  "ob_OELK_EPS_Factor_Control"
  ob_In_convert84/1 -> ob_In_terminator84/1  "ob_OELK_EPS_ELK_Control"
  ob_In_convert85/1 -> ob_In_terminator85/1  "ob_OELK_ELK_VehicleLaneDisp"
  ob_In_convert86/1 -> ob_In_terminator86/1  "ob_OELK_ELK_ELKSts"
  ob_In_convert87/1 -> ob_In_terminator87/1  "ob_OELK_SignalTStamp"
  ob_In_convert88/1 -> ob_In_terminator88/1  "ob_OICAB_PathQI"
  ob_In_convert89/1 -> ob_In_terminator89/1  "ob_OICAB_SignalTStamp"
  ob_In_convert90/1 -> ob_In_terminator90/1  "ob_OICAB_ICAB2HMI"
  ob_In_convert91/1 -> ob_In_terminator91/1  "ob_OICAB_SteerAngleCmd"
  ob_In_convert92/1 -> ob_In_terminator92/1  "ob_OICAB_ICAMode"
  ob_In_convert93/1 -> ob_In_terminator93/1  "ob_OICAB_ICAState"
  ob_In_convert94/1 -> ob_In_terminator94/1  "ob_OICAD_DecionState"
  ob_In_convert95/1 -> ob_In_terminator95/1  "ob_OICAD_DecionCMD"
  ob_In_convert96/1 -> ob_In_terminator96/1  "ob_OICAD_LCRecommend"
  ob_In_convert97/1 -> ob_In_terminator97/1  "ob_OICAD_SignalTStamp"
  ob_In_convert117/1 -> ob_In_terminator117/1  "ob_OIMAP_EPS_LKA_State"
  ob_In_convert118/1 -> ob_In_terminator118/1  "ob_OIMAP_ESC_LonAcc"
  ob_In_convert119/1 -> ob_In_terminator119/1  "ob_OIMAP_obj_id"
  ob_In_convert120/1 -> ob_In_terminator120/1  "ob_OIMAP_obj_pos_x"
  ob_In_convert121/1 -> ob_In_terminator121/1  "ob_OIMAP_ESC_Veh_Standstill"
  ob_In_convert122/1 -> ob_In_terminator122/1  "ob_OIMAP_L0_C0"
  ob_In_convert123/1 -> ob_In_terminator123/1  "ob_OIMAP_L0_C1"
  ob_In_convert124/1 -> ob_In_terminator124/1  "ob_OIMAP_L0_C2"
  ob_In_convert125/1 -> ob_In_terminator125/1  "ob_OIMAP_L0_C3"
  ob_In_convert126/1 -> ob_In_terminator126/1  "ob_OIMAP_R0_C0"
  ob_In_convert127/1 -> ob_In_terminator127/1  "ob_OIMAP_R0_C1"
  ob_In_convert128/1 -> ob_In_terminator128/1  "ob_OIMAP_R0_C2"
  ob_In_convert129/1 -> ob_In_terminator129/1  "ob_OIMAP_R0_C3"
  [ICA_EPS] -> Index Vector2/10
  IMAPve_d_APA_AutoPark_WorkSt/1 -> Gain6/1
  Data Type Conversion32/1 -> Bus_IMAP/14  "IMAPve_d_APA_AutoPark_WorkSt"
  Data Type Conversion37/1 -> Bus_ACCS/21  "ACCSve_d_ACC_ISLCState_convert"
  Data Type Conversion38/1 -> Bus_ACCS/22  "ACCSve_d_ACC_ISLCDriverRemind_convert"
  ACCSve_d_ACC_ISLCState/1 -> Gain1/1
  Data Type Conversion43/1 -> ob_In_terminator149/1  "ob_OACC_ACC_ISLCState"
  ACCSve_d_ACC_ISLCDriverRemind/1 -> Gain/1
  Data Type Conversion44/1 -> ob_In_terminator150/1  "ob_OACC_ACC_ISLCDriverRemind"
  Data Type Conversion45/1 -> ob_In_terminator151/1  "ob_OIMAP_APA_AutoPark_WorkSt"
  Gain/1 -> Data Type Conversion44/1, Data Type Conversion38/1
  Gain1/1 -> Data Type Conversion43/1, Data Type Conversion37/1
  Gain6/1 -> Data Type Conversion45/1, Data Type Conversion32/1
  Gain7/1 -> ob_In_convert140/1, Data Type Conversion88/1
  Gain8/1 -> ob_In_convert139/1, Data Type Conversion87/1
  Gain9/1 -> ob_In_convert142/1, Data Type Conversion179/1
  Gain10/1 -> ob_In_convert141/1, Data Type Conversion178/1
  Gain11/1 -> ob_In_convert144/1, Data Type Conversion182/1
  Gain12/1 -> ob_In_convert143/1, Data Type Conversion180/1
  [ICA_Input] -> Subsystem/7(Input_ICA)
  [JA_Input] -> Subsystem/3(Input_JABS)
  [ESA_Input] -> Subsystem/6(Input_ESAS)
  [ELK_Input] -> Subsystem/5(Input_ELKS)
  [AEB_Input] -> Subsystem/2(Input_AEBS)
  [ACC_Input] -> Subsystem/1(Input_ACCS)
  [LKA_Input] -> Subsystem/4(Input_LKAS)
  [FD_Input] -> Subsystem/8(Input_FDMM)
  [IMAP_Input] -> Subsystem/9(Input_IMAP)
  Subsystem6/1(Out1) -> ob_convert65/1, OMAPve_y_ADAS_ELKPopupMessage/1
  ob_convert65/1 -> ob_terminator64/1  "ob_OMAPve_y_ADAS_ELKPopupMessage"
  Subsystem3/7(Out7) -> ob_convert34/1, OMAPve_y_ADAS_AEBState/1
  Subsystem6/10(Out10) -> ob_convert61/1, OMAPve_y_ADAS_JAFaultSt/1
  Constant7/1 -> ob_convert172/1
  Subsystem3/10(Out10) -> ob_convert37/1, OMAPve_y_ADAS_HapticAlarmReq/1
  Bus Selector1/12 -> ?  "<OMAPve_y_Haptic_Alarm_1>"
  Subsystem6/9(Out9) -> ob_convert72/1, OMAPve_y_ADAS_TurnLightsCommand/1
  Data Type Conversion33/1 -> Bus Creator/1  "ESASve_y_ESA_State_convert"
  Data Type Conversion34/1 -> Bus Creator/2  "ESASve_g_ESA_SWA_CMD_convert"
  ESASve_g_ESA_SWA_CMD/1 -> Data Type Conversion46/1, Data Type Conversion34/1
  ESASve_g_EPS_Factor_Control/1 -> Data Type Conversion47/1, Data Type Conversion35/1
  Data Type Conversion35/1 -> Bus Creator/3  "ESASve_g_EPS_Factor_Control_convert"
  Data Type Conversion36/1 -> Bus Creator/4  "ESASve_y_ESA_FaultSt_convert"
  ESASve_y_ESA_FaultSt/1 -> Data Type Conversion48/1, Data Type Conversion36/1
  ESASve_y_ESARequest/1 -> Data Type Conversion49/1, Data Type Conversion39/1
  Data Type Conversion39/1 -> Bus Creator/5  "ESASve_y_ESARequest_convert"
  Data Type Conversion40/1 -> Bus Creator/6  "ESASve_y_ESATorqueReq_convert"
  ESASve_y_ESATorqueReq/1 -> Data Type Conversion50/1, Data Type Conversion40/1
  Data Type Conversion41/1 -> Bus Creator/7  "ESASve_y_LKAActivation_convert"
  ESASve_y_LKAActivation/1 -> Data Type Conversion51/1, Data Type Conversion41/1
  Default_EMS/1(Default_EMS) -> Index Vector/11, Index Vector/2
  Data Type Conversion42/1 -> ob_In_terminator98/1  "ob_OESA_ESA_State"
  Data Type Conversion46/1 -> ob_In_terminator99/1  "ob_OESA_ESA_SWA_CMD"
  Data Type Conversion47/1 -> ob_In_terminator100/1  "ob_OESA_EPS_Factor_Control"
  Data Type Conversion48/1 -> ob_In_terminator101/1  "ob_OESA_ESA_FaultSt"
  Data Type Conversion49/1 -> ob_In_terminator102/1  "ob_OESA_ESARequest"
  Data Type Conversion50/1 -> ob_In_terminator103/1  "ob_OESA_ESATorqueReq"
  Data Type Conversion51/1 -> ob_In_terminator104/1  "ob_OESA_LKAActivation"
  Default_IC/1(Default_IC) -> Index Vector3/11, Index Vector3/2
  [ELK_IC] -> Index Vector3/8
  [ESA_IC] -> Index Vector3/9
  [ICA_IC] -> Index Vector3/10
  [ob_AEBarbJADecType] -> CAN Pack/3
  [ob_isLowACCandLowAEB] -> CAN Pack/5
  [ob_isJAorDeepAEB] -> CAN Pack/4
  CAN Pack/1 -> CAN Unpack/1
  CAN Unpack/2 -> OMAPve_g_ob019L_100/1
  [ob_AEBarbJADecReq] -> CAN Pack/1
  [ob_AEBarbJADecSet] -> CAN Pack/2
  ACCSve_d_ACCMessagePrompt/1 -> Data Type Conversion53/1, Data Type Conversion52/1
  Data Type Conversion52/1 -> Bus_ACCS/23  "ACCSve_d_ACCMessagePrompt_convert"
  Data Type Conversion53/1 -> ob_In_terminator105/1  "ob_OACC_ACCMessagePrompt"
  Bus Selector/3 -> Subsystem2/1(OMAPve_g_ACCTqReq_1)  "<OMAPve_g_ACCTqReq_1>"
  Bus Selector/4 -> Subsystem2/2(OMAPve_y_Powertrain_torquewheel_request_1)  "<OMAPve_y_Powertrain_torquewheel_request_1>"
  Bus Selector/5 -> Subsystem2/3(OMAPve_g_TminUp_or_downGear_1)  "<OMAPve_g_TminUp_or_downGear_1>"
  Bus Selector/7 -> Subsystem2/4(OMAPve_y_Function_Acc_status_1)  "<OMAPve_y_Function_Acc_status_1>"
  Bus Selector1/1 -> Subsystem3/1(OMAPve_g_Deceleration_setpoint_device_1)  "<OMAPve_g_Deceleration_setpoint_device_1>"
  Bus Selector1/2 -> Subsystem3/2(OMAPve_y_MDD_Decelerationcontrol_request_1)  "<OMAPve_y_MDD_Decelerationcontrol_request_1>"
  Bus Selector1/3 -> Subsystem3/3(OMAPve_y_Prefill_request_1)  "<OMAPve_y_Prefill_request_1>"
  Bus Selector1/4 -> Subsystem3/4(OMAPve_y_ADAS_ESCDriveOff)  "<OMAPve_y_ADAS_ESCDriveOff>"
  Bus Selector1/5 -> Subsystem3/5(OMAPve_y_ADAS_ESCHoldReq)  "<OMAPve_y_ADAS_ESCHoldReq>"
  Bus Selector1/6 -> Subsystem3/6(OMAPve_y_MDD_deceleration_type_1)  "<OMAPve_y_MDD_deceleration_type_1>"
  Bus Selector1/8 -> Subsystem1/1(In1)  "<OMAPve_y_AEB_Status_1>"
  Bus Selector1/9 -> Subsystem3/8(OMAPve_y_Decel_Request_1)  "<OMAPve_y_Decel_Request_1>"
  Bus Selector1/10 -> Subsystem3/9(OMAPve_y_AEB_Braking_progress_1)  "<OMAPve_y_AEB_Braking_progress_1>"
  ob_convert172/1 -> Subsystem3/10(OMAPve_y_Haptic_Alarm_1)  "OMAPve_y_Haptic_Alarm_1"
  Bus Selector1/13 -> Subsystem3/11(OMAPve_y_ADAS_ACCRequestEPB)  "<OMAPve_y_ADAS_ACCRequestEPB>"
  Subsystem1/1(Out1) -> Subsystem3/7(OMAPve_y_AEB_Status_1)  "OMAPve_y_AEB_Status_1"
  Bus Selector2/2 -> Subsystem4/1(OMAPve_y_General_state_of_LKA_function3F2_2)  "<OMAPve_y_General_state_of_LKA_function3F2_2>"
  Bus Selector2/3 -> Subsystem4/2(OMAPve_g_Coefficient_toregulate_EPS_2)  "<OMAPve_g_Coefficient_toregulate_EPS_2>"
  Bus Selector2/4 -> Subsystem4/3(OMAPve_g_Column_angle_setpoint3F2_2)  "<OMAPve_g_Column_angle_setpoint3F2_2>"
  Bus Selector2/5 -> Subsystem4/4(OMAPve_y_Permit_to_know_if_LKA_or_LPA3F2_2)  "<OMAPve_y_Permit_to_know_if_LKA_or_LPA3F2_2>"
  Bus Selector2/6 -> Subsystem4/5(OMAPve_y_ADAS_ESAState_2)  "<OMAPve_y_ADAS_ESAState_2>"
  Bus Selector2/7 -> Subsystem4/6(OMAPve_g_ADAS_ESATorqueReq_2)  "<OMAPve_g_ADAS_ESATorqueReq_2>"
  Bus Selector2/8 -> Subsystem4/7(OMAPve_y_ADAS_ESARequest_2)  "<OMAPve_y_ADAS_ESARequest_2>"
  Bus Selector4/3 -> Subsystem8/1(OMAPve_y_TYPE_RAPPORT_2)  "<OMAPve_y_TYPE_RAPPORT_2>"
  Bus Selector3/1 -> Subsystem6/1(OMAPve_y_ADAS_ELKPopupMessage_2)  "<OMAPve_y_ADAS_ELKPopupMessage_2>"
  Bus Selector3/2 -> Subsystem6/2(OMAPve_y_ADAS_ESAFaultSt_2)  "<OMAPve_y_ADAS_ESAFaultSt_2>"
  Bus Selector3/3 -> Subsystem6/3(OMAPve_y_ADAS_HWAMode_2)  "<OMAPve_y_ADAS_HWAMode_2>"
  Bus Selector3/4 -> Subsystem6/4(OMAPve_y_ADAS_HWATurnOnIndicator_2)  "<OMAPve_y_ADAS_HWATurnOnIndicator_2>"
  Bus Selector3/5 -> Subsystem6/5(OMAPve_y_ADAS_HWAActionSts_2)  "<OMAPve_y_ADAS_HWAActionSts_2>"
  Bus Selector3/6 -> Subsystem6/6(OMAPve_y_ADAS_LightControlValid_2)  "<OMAPve_y_ADAS_LightControlValid_2>"
  Bus Selector3/7 -> Subsystem6/7(OMAPve_y_ADAS_ISLCState_2)  "<OMAPve_y_ADAS_ISLCState_2>"
  Bus Selector3/8 -> Subsystem6/8(OMAPve_y_ADAS_ISLCDriverRemind_2)  "<OMAPve_y_ADAS_ISLCDriverRemind_2>"
  Bus Selector3/9 -> Subsystem6/9(OMAPve_y_ADAS_TurnLightsCommand_2)  "<OMAPve_y_ADAS_TurnLightsCommand_2>"
  Bus Selector3/10 -> Subsystem6/10(OMAPve_y_ADAS_JAFaultSt_2)  "<OMAPve_y_ADAS_JAFaultSt_2>"
  Bus Selector3/12 -> Subsystem6/11(OMAPve_y_ACC_DesiredHeadway_Display_2)  "<OMAPve_y_ACC_DesiredHeadway_Display_2>"
  Bus Selector3/13 -> Subsystem6/12(OMAPve_y_ACC_DesiredHeadway_Icon_Basic_2)  "<OMAPve_y_ACC_DesiredHeadway_Icon_Basic_2>"
  Bus Selector3/14 -> Subsystem6/13(OMAPve_y_ACC_Desired_Set_Speed_2)  "<OMAPve_y_ACC_Desired_Set_Speed_2>"
  Bus Selector3/15 -> Subsystem6/14(OMAPve_y_ACC_Set_Speed_Display_2)  "<OMAPve_y_ACC_Set_Speed_Display_2>"
  Bus Selector3/16 -> Subsystem6/15(OMAPve_y_ACC_Vehicle_Icon_Display_2)  "<OMAPve_y_ACC_Vehicle_Icon_Display_2>"
  Bus Selector3/17 -> Subsystem6/16(OMAPve_y_RVVACC_Vehiclespeed_request_type_2)  "<OMAPve_y_RVVACC_Vehiclespeed_request_type_2>"
  Bus Selector3/18 -> Subsystem6/17(OMAPve_y_ACC_Pop_Up_Message_2)  "<OMAPve_y_ACC_Pop_Up_Message_2>"
  Bus Selector3/19 -> Subsystem6/18(OMAPve_y_AEB_Alert_Req_2)  "<OMAPve_y_AEB_Alert_Req_2>"
  Bus Selector3/20 -> Subsystem6/19(OMAPve_y_AEB_Fault_Status_2)  "<OMAPve_y_AEB_Fault_Status_2>"
  Bus Selector3/21 -> Subsystem6/20(OMAPve_y_AEB_Switch_Status_2)  "<OMAPve_y_AEB_Switch_Status_2>"
  Bus Selector3/22 -> Subsystem6/21(OMAPve_y_AEB_tips_2)  "<OMAPve_y_AEB_tips_2>"
  Bus Selector3/25 -> Subsystem6/22(OMAPve_y_Hands_off_warning_2)  "<OMAPve_y_Hands_off_warning_2>"
  Bus Selector3/26 -> Subsystem6/23(OMAPve_y_HMI_Popup_Status_2)  "<OMAPve_y_HMI_Popup_Status_2>"
  Bus Selector3/27 -> Subsystem6/24(OMAPve_y_Vehicle_Lane_Display_2)  "<OMAPve_y_Vehicle_Lane_Display_2>"
  Bus Selector3/28 -> Subsystem6/25(OMAPve_y_LDW_Flag_2)  "<OMAPve_y_LDW_Flag_2>"
  Bus Selector3/29 -> Subsystem6/26(OMAPve_y_LDW_Status_Display_2)  "<OMAPve_y_LDW_Status_Display_2>"
  Bus Selector3/30 -> Subsystem6/27(OMAPve_y_LKA_Mode_from_Camera_2)  "<OMAPve_y_LKA_Mode_from_Camera_2>"
  Bus Selector3/31 -> Subsystem6/28(OMAPve_y_LKA_Status_Display_2)  "<OMAPve_y_LKA_Status_Display_2>"
  Bus Selector3/32 -> Subsystem6/29(OMAPve_y_LKA_Switch_State_2)  "<OMAPve_y_LKA_Switch_State_2>"
  Bus Selector3/34 -> Subsystem6/30(OMAPve_y_ADAS_ELKSts_2)  "<OMAPve_y_ADAS_ELKSts_2>"
  Bus Selector3/35 -> Subsystem6/31(OMAPve_y_ICA_HMI_Txt_Disp_2)  "<OMAPve_y_ICA_HMI_Txt_Disp_2>"
  Bus Selector3/36 -> Subsystem6/32(OMAPve_y_TJA_status_icon_2)  "<OMAPve_y_TJA_status_icon_2>"
  ob_convert178/1 -> Subsystem7/3(OMAPve_y_ADAS_State1)  "OMAPve_y_ADAS_State1"
  ob_convert165/1 -> Subsystem7/2(OMAPve_y_ADAS_LCAPopupMessage1)  "OMAPve_y_ADAS_LCAPopupMessage1"
  ob_convert164/1 -> Subsystem7/1(OMAPve_y_ADAS_LCAStatusDisplay1)  "OMAPve_y_ADAS_LCAStatusDisplay1"
